simulink model "MICRORRED"  (R2018a)
settings: Solver=FixedStepDiscrete  StartTime=0.0  StopTime=0.7  FixedStep=1/(60*32)  RelTol=1e-3  EnableMultiTasking=on
InitFcn:
  | close
  | clear
  | clc
  | Ts=1/(60*32);
  | run script_client_3_inicio_ti.m
  | set_param('MICRORRED/EMISOR-RECEPTOR/TCP_IP_RX3/ESCRITURA', 'Value','0');
  | set_param('MICRORRED/EMISOR-RECEPTOR/TCP_IP_RX3/RETARDO', 'Value','0');
StopFcn:
  | %run script_graficas.m
undefined symbols (not defined in the file or in its folder): DiscIntNeverNeededParam, Int, Ip1, man, Vuc
libraries: powerlib x15, simulink x6, libreria_medidores3 x2, libreria_comunicaciones_red3 x1
(part 1 of 2)
settings Model: SnapshotInterval=1  Creator=Juan Antonio Ocampo  LastModifiedBy=ana-n
settings DataIOCC: LimitDataPoints=on
settings OptimizationCC: LifeSpan=inf
settings DebuggingCC: AllowSymbolicDim=off  SFUnexpectedBacktrackingDiag=warning  SFNoUnconditionalDefaultTransitionDiag=warning  SFExecutionAtInitializationDiag=none
settings ModelReferenceCC: PropagateSignalLabelsOutOfModel=off
settings CodeAppCC: StateflowObjectComments=on
settings GRTTargetCC: TargetLangStandard=C89/C90 (ANSI)
settings ConfigComp: CovMetricSettings=dw  CovHtmlReporting=on  CovSaveCumulativeToWorkspaceVar=on  CovSaveSingleToWorkspaceVar=on  CovExternalEMLEnable=off
settings SimscapeCC: SimscapeNormalizeSystem=off

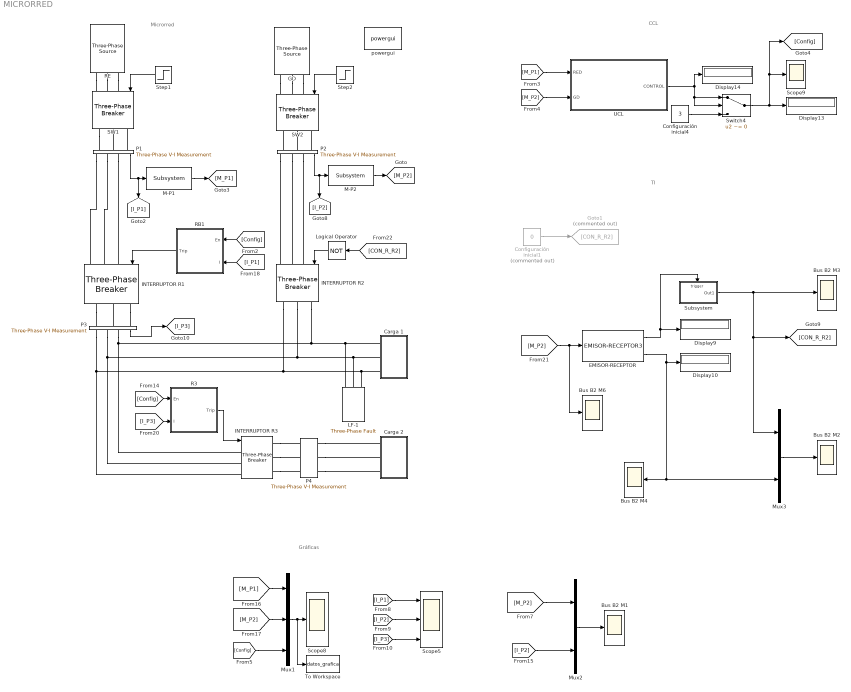
== system MICRORRED ==
  note: Microrred
  note: Gráficas
  note: TI
  note: CCL
  "               LF-1" : powerlib/Elements/Three-Phase Fault  InitialStates=0  FaultA=on  FaultB=on  FaultC=on  GroundFault=on  SwitchTimes=0.4  External=off  SwitchStatus=NaN  FaultResistance=50  GroundResistance=400  SnubberResistance=1e6  SnubberCapacitance=inf  Measurements=Fault currents
  Bus B2 M{1..4,6} (5 alike) : Scope
  Carga 1 : Subsystem
  Carga 2 : Subsystem
  Configuración inicial1 : Constant  Commented=on  Value=0
  Configuración inicial4 : Constant  Value=3
  Display{9..10,13..14} (4 alike) : Display
  EMISOR-RECEPTOR : libreria_comunicaciones_red3/EMISOR-RECEPTOR3  SystemSampleTime=-1
      link override TCP_IP_RX3/ESCRITURA: Value=client_1.dato_lectura
      link override TCP_IP_RX3/RETARDO: Value=e
  GD : powerlib/Electrical Sources/Three-Phase Source  InternalConnection=Yg  VoltagePhases=off  Voltage=13200  PhaseAngle=0  Voltage_phases=[25e3 25e3 25e3]/sqrt(3)  PhaseAngles_phases=[0 -120 +120]  Frequency=60  NonIdealSource=on  SpecifyImpedance=on  Resistance=25^2/1000/10  Inductance=25^2/1000/377  ShortCircuitLevel=100e6  BaseVoltage=13200  XRratio=10  BusType=swing  Pref=1000  Qref=0  Prefabc=[10e3, 10e3, 10e3]  Qrefabc=[0, 0, 0]  Qmin=-inf  Qmax=inf
  Goto1 : Goto  Commented=on  GotoTag=CON_R_R2
  INTERRUPTOR R1 : powerlib/Elements/Three-Phase Breaker  InitialState=closed  SwitchA=on  SwitchB=on  SwitchC=on  SwitchTimes=[20]  External=on  BreakerResistance=0.0000001  SnubberResistance=1e6  SnubberCapacitance=inf  Measurements=None
      link override Breaker A: Measurements=None
      link override Breaker B: Measurements=None
      link override Breaker C: Measurements=None
  INTERRUPTOR R2 : powerlib/Elements/Three-Phase Breaker  InitialState=closed  SwitchA=on  SwitchB=on  SwitchC=on  SwitchTimes=[20]  External=on  BreakerResistance=0.0000001  SnubberResistance=1e6  SnubberCapacitance=inf  Measurements=None
      link override Breaker A: Measurements=None
      link override Breaker B: Measurements=None
      link override Breaker C: Measurements=None
  INTERRUPTOR R3 : powerlib/Elements/Three-Phase Breaker  InitialState=closed  SwitchA=on  SwitchB=on  SwitchC=on  SwitchTimes=[20]  External=on  BreakerResistance=0.0000001  SnubberResistance=1e6  SnubberCapacitance=inf  Measurements=None
      link override Breaker A: Measurements=None
      link override Breaker B: Measurements=None
      link override Breaker C: Measurements=None
  Logical Operator : Logic  Operator=NOT  AllPortsSameDT=off  OutDataTypeStr=fixdt(1,16)
  M-P1 : libreria_medidores3/Subsystem  SystemSampleTime=-1
  M-P2 : libreria_medidores3/Subsystem  SystemSampleTime=-1
  Mux1 : Mux  Inputs=3
  Mux2 : Mux  Inputs=2
  Mux3 : Mux  Inputs=2
  P1 : powerlib/Measurements/Three-Phase V-I Measurement  VoltageMeasurement=no  SetLabelV=off  LabelV=V_P1  Vpu=off  VpuLL=off  CurrentMeasurement=yes  SetLabelI=off  LabelI=I_P1  Ipu=off  Pbase=100e6  Vbase=500e3  OutputType=Complex  PhasorSimulation=off  PSBequivalent=0
  P2 : powerlib/Measurements/Three-Phase V-I Measurement  VoltageMeasurement=no  SetLabelV=on  LabelV=V_P2  Vpu=off  VpuLL=off  CurrentMeasurement=yes  SetLabelI=off  LabelI=I_P2  Ipu=off  Pbase=100e6  Vbase=500e3  OutputType=Complex  PhasorSimulation=off  PSBequivalent=0
  P3 : powerlib/Measurements/Three-Phase V-I Measurement  VoltageMeasurement=no  SetLabelV=off  LabelV=V_P1  Vpu=off  VpuLL=off  CurrentMeasurement=yes  SetLabelI=off  LabelI=I_P1  Ipu=off  Pbase=100e6  Vbase=500e3  OutputType=Complex  PhasorSimulation=off  PSBequivalent=0
  P4 : powerlib/Measurements/Three-Phase V-I Measurement  VoltageMeasurement=phase-to-ground  SetLabelV=on  LabelV=V_P4  Vpu=off  VpuLL=off  CurrentMeasurement=yes  SetLabelI=on  LabelI=I_P4  Ipu=off  Pbase=100e6  Vbase=500e3  OutputType=Complex  PhasorSimulation=off  PSBequivalent=0
  R3 : Subsystem  mask(Proteccion de Sobrecorriente multitopologia){menu=3, TCpopup1=IEC Standard Inverse, k1=0.14, alpha1=0.02, B1=0, PS1=1.15, TMS1=0.04, Tins1=0.05, Esc1=3, TCpopup2=IEC Standard Inverse, k2=0.14, alpha2=0.02, B2=0, PS2=1.15, TMS2=0.03, Tins2=0.05, Esc2=3, TCpopup3=IEC Standard Inverse, k3=0.14, alpha3=0.02, B3=0, PS3=1.15, TMS3=0.01, Tins3=0.03, Esc3=3, Vp=25, Vs=25, F=60}
      mask prompts: menu "Numero de Topologias"; TCpopup1 "Caracteristica de Disparo"; k1 "k"; alpha1 "alpha"; B1 "B"; PS1 "Seteo disparo(PS)/Seteo inferior(I>)"; TMS1 "Multiplicador de Tiempo"; Tins1 "Tins"; Esc1 "Escala"; TCpopup2 "Caracteristica de Disparo"; k2 "k"; alpha2 "alpha"; B2 "B"; PS2 "Seteo disparo(PS)/Seteo inferior(I>)"; TMS2 "Multiplicador de tiempo"; Tins2 "Tins"; Esc2 "Escala"; TCpopup3 "Caracteristica de Disparo"; k3 "k"; alpha3 "alpha"; B3 "B"; PS3 "Seteo disparo(PS)/Seteo inferior(I>)"; TMS3 "Multiplicador de Tiempo"; Tins3 "Tins"; Esc3 "Escala"; Vp "Primario CT"; Vs "Secundario CT"; F "Frecuencia"
      mask help: Proteccion de Sobrecorriente con tres topologias internas controladas por una señal de control externa.
      mask init:
      | warning('off','Simulink:Masking:Invalid_Visible_Flag')
      mask TypeOptions menu: 1 | 2 | 3
      mask Callback menu:
      | h = getSimulinkBlockHandle(gcb);
      | menu1 = get_param(h,'menu');
      | if strcmp(menu1,num2str(1))
      |     set_param(h,'MaskVisibilities',{'on',...
      |         'on','on','on','on','on','on','on','on',...%proteccion 1 activa
      |         'off','off','off','off','off','off','off','off',...%proteccion 2 desactivada
      |         'off','off','off','off','off','off','off','off',...%proteccion 3 desactivada
      |         'on','on','on'});%Otros parametros activados
      |     Int=1;
      | elseif strcmp(menu1,num2str(2))
      |  set_param(h,'MaskVisibilities',{'on',...
      |         'on','on','on','on','on','on','on','on',...%proteccion 1 activa
      |         'on','on','on','on','on','on','on','on',...%proteccion 2 activa
      |         'off','off','off','off','off','off','off','off',...%proteccion 3 desactivada
      |         'on','on','on'});%Otros parametros activados
      |     Int=2;
      | else
      | set_param(h,'MaskVisibilities',{'on',...
      |         'on','on','on','on','on','on','on','on',...%proteccion 1 activa
      |         'on','on','on','on','on','on','on','on',...%proteccion 2 activa
      |         'on','on','on','on','on','on','on','on',...%proteccion 3 desactivada
      |         'on','on','on'});%Otros parametros activados
      |     Int=3;
      | end
      mask TypeOptions TCpopup1: IEC Standard Inverse | IEC Very Inverse | IEC Long Time Inverse | IEC Extremely Inverse | IEC Ultra Inverse | IEEE Moderately Inverse | IEEE Very Inverse | IEEE Extremely Inverse
      mask Callback TCpopup1:
      | switch(get_param(gcb,'TCpopup1'))
      |     case 'IEC Standard Inverse'
      |         set_param(gcb,'k1','0.14');
      |         set_param(gcb,'alpha1','0.02');
      |         set_param(gcb,'B1','0');
      |     case 'IEC Very Inverse'
      |         set_param(gcb,'k1','13.5');
      |         set_param(gcb,'alpha1','1');
      |         set_param(gcb,'B1','0');
      |     case 'IEC Long Time Inverse'
      |         set_param(gcb,'k1','120');
      |         set_param(gcb,'alpha1','1');
      |         set_param(gcb,'B1','0');
      |     case 'IEC Extremely Inverse'
      |         set_param(gcb,'k1','80');
      |         set_param(gcb,'alpha1','2');
      |         set_param(gcb,'B1','0');
      |     case 'IEC Ultra Inverse'
      |         set_param(gcb,'k1','315.2');
      |         set_param(gcb,'alpha1','2.5');
      |         set_param(gcb,'B1','0');
      |     case 'IEEE Moderately Inverse'
      |         set_param(gcb,'k1','0.0515');
      |         set_param(gcb,'alpha1','0.02');
      |         set_param(gcb,'B1','0.114');
      |     case 'IEEE Very Inverse'
      |         set_param(gcb,'k1','19.61');
      |         set_param(gcb,'alpha1','2');
      |         set_param(gcb,'B1','0.491');
      |     case 'IEEE Extremely Inverse'
      |         set_param(gcb,'k1','28.2');
      |         set_param(gcb,'alpha1','2');
      |         set_param(gcb,'B1','0.1217');
      | end
      | % Plotting IDMT Curve
      | clf('reset')
      | TMS = str2num(get_param(gcb,'TMS1'));
      | Vp = str2num(get_param(gcb,'Vp'));
      | PS=str2num(get_param(gcb,'PS1'));
      | k = str2num(get_param(gcb,'k1'));
      | alpha = str2num(get_param(gcb,'alpha1'));
      | B = str2num(get_param(gcb,'B1'));
      | Esc = str2num(get_param(gcb,'Esc1'));
      | Tins = str2num(get_param(gcb,'Tins1'));
      | I = [1.1:0.1:Esc];
      | I1=[Esc,Esc:0.1:30];
      | y=((k./((I.^alpha)-1))+B)*TMS;
      | Tin=[((k./((Esc.^alpha)-1))+B)*TMS,ones(1,length(I1)-1)*Tins];
      | loglog(I,y,'b');
      | hold on
      | loglog(I1,Tin,'b');
      | set(gcf, 'Position', [200 150 300 500]);
      | switch(get_param(gcb,'TCpopup1'))
      |     case 'IEC Standard Inverse'
      |         title('IEC Standard Inverse');
      |     case 'IEC Very Inverse'
      |         title('IEC Very Inverse');
      |     case 'IEC Long Time Inverse'
      |         title('IEC Long Time Inverse');
      |     case 'IEC Extremely Inverse'
      |         title('IEC Extremely Inverse');
      |      case 'IEC Ultra Inverse'
      |         title('IEC Ultra Inverse');
      |     case 'IEEE Moderately Inverse'
      |         title('IEEE Moderately Inverse');
      |     case 'IEEE Very Inverse'
      |         title('IEEE Very Inverse');
      |     case 'IEEE Extremely Inverse'
      |         title('IEEE Extremely Inverse');
      | end
      | ymax=10^ceil(log10(max(y)));
      | set(gca, 'XTick',[1:10 20]);
      | set(gca, 'YTick',[0 ymax/1000 ymax/500 ymax/200 ymax/100 ymax/50 ymax/20 ymax/10 ymax/5 ymax/2 ymax]);
      | xlim([0.9 30]);
      | ylim([0.01 ymax]);
      | xlabel(['Corriente multiplicada por Ipick-up(' num2str(PS*Vp) 'A)']);
      | ylabel('Tiempo de Operacion (Seg)');
      | grid on;
      | set(gca, 'color',[0.9608 0.9608 0.937]);
      | set(gca, 'gridcolor',[0 0.6902 0.3137]);
      mask Callback PS1:
      | % Plotting IDMT Curve
      | clf('reset')
      | TMS = str2num(get_param(gcb,'TMS1'));
      | Vp = str2num(get_param(gcb,'Vp'));
      | PS=str2num(get_param(gcb,'PS1'));
      | k = str2num(get_param(gcb,'k1'));
      | alpha = str2num(get_param(gcb,'alpha1'));
      | B = str2num(get_param(gcb,'B1'));
      | Esc = str2num(get_param(gcb,'Esc1'));
      | Tins = str2num(get_param(gcb,'Tins1'));
      | I = [1.1:0.1:Esc];
      | I1=[Esc,Esc:0.1:30];
      | y=((k./((I.^alpha)-1))+B)*TMS;
      | Tin=[((k./((Esc.^alpha)-1))+B)*TMS,ones(1,length(I1)-1)*Tins];
      | loglog(I,y,'b');
      | hold on
      | loglog(I1,Tin,'b');
      | set(gcf, 'Position', [200 150 300 500]);
      | switch(get_param(gcb,'TCpopup1'))
      |     case 'IEC Standard Inverse'
      |         title('IEC Standard Inverse');
      |     case 'IEC Very Inverse'
      |         title('IEC Very Inverse');
      |     case 'IEC Long Time Inverse'
      |         title('IEC Long Time Inverse');
      |     case 'IEC Extremely Inverse'
      |         title('IEC Extremely Inverse');
      |      case 'IEC Ultra Inverse'
      |         title('IEC Ultra Inverse');
      |     case 'IEEE Moderately Inverse'
      |         title('IEEE Moderately Inverse');
      |     case 'IEEE Very Inverse'
      |         title('IEEE Very Inverse');
      |     case 'IEEE Extremely Inverse'
      |         title('IEEE Extremely Inverse');
      | end
      | ymax=10^ceil(log10(max(y)));
      | set(gca, 'XTick',[1:10 20]);
      | set(gca, 'YTick',[0 ymax/1000 ymax/500 ymax/200 ymax/100 ymax/50 ymax/20 ymax/10 ymax/5 ymax/2 ymax]);
      | xlim([0.9 30]);
      | ylim([0.01 ymax]);
      | xlabel(['Corriente multiplicada por Ipick-up(' num2str(PS*Vp) 'A)']);
      | ylabel('Tiempo de Operacion (Seg)');
      | grid on;
      | set(gca, 'color',[0.9608 0.9608 0.937]);
      | set(gca, 'gridcolor',[0 0.6902 0.3137]);
      mask Callback TMS1:
      | % Plotting IDMT Curve
      | clf('reset')
      | TMS = str2num(get_param(gcb,'TMS1'));
      | Vp = str2num(get_param(gcb,'Vp'));
      | PS=str2num(get_param(gcb,'PS1'));
      | k = str2num(get_param(gcb,'k1'));
      | alpha = str2num(get_param(gcb,'alpha1'));
      | B = str2num(get_param(gcb,'B1'));
      | Esc = str2num(get_param(gcb,'Esc1'));
      | Tins = str2num(get_param(gcb,'Tins1'));
      | I = [1.1:0.1:Esc];
      | I1=[Esc,Esc:0.1:30];
      | y=((k./((I.^alpha)-1))+B)*TMS;
      | Tin=[((k./((Esc.^alpha)-1))+B)*TMS,ones(1,length(I1)-1)*Tins];
      | loglog(I,y,'b');
      | hold on
      | loglog(I1,Tin,'b');
      | set(gcf, 'Position', [200 150 300 500]);
      | switch(get_param(gcb,'TCpopup1'))
      |     case 'IEC Standard Inverse'
      |         title('IEC Standard Inverse');
      |     case 'IEC Very Inverse'
      |         title('IEC Very Inverse');
      |     case 'IEC Long Time Inverse'
      |         title('IEC Long Time Inverse');
      |     case 'IEC Extremely Inverse'
      |         title('IEC Extremely Inverse');
      |      case 'IEC Ultra Inverse'
      |         title('IEC Ultra Inverse');
      |     case 'IEEE Moderately Inverse'
      |         title('IEEE Moderately Inverse');
      |     case 'IEEE Very Inverse'
      |         title('IEEE Very Inverse');
      |     case 'IEEE Extremely Inverse'
      |         title('IEEE Extremely Inverse');
      | end
      | ymax=10^ceil(log10(max(y)));
      | set(gca, 'XTick',[1:10 20]);
      | set(gca, 'YTick',[0 ymax/1000 ymax/500 ymax/200 ymax/100 ymax/50 ymax/20 ymax/10 ymax/5 ymax/2 ymax]);
      | xlim([0.9 30]);
      | ylim([0.01 ymax]);
      | xlabel(['Corriente multiplicada por Ipick-up(' num2str(PS*Vp) 'A)']);
      | ylabel('Tiempo de Operacion (Seg)');
      | grid on;
      | set(gca, 'color',[0.9608 0.9608 0.937]);
      | set(gca, 'gridcolor',[0 0.6902 0.3137]);
      mask Callback Tins1:
      | % Plotting IDMT Curve
      | clf('reset')
      | TMS = str2num(get_param(gcb,'TMS1'));
      | Vp = str2num(get_param(gcb,'Vp'));
      | PS=str2num(get_param(gcb,'PS1'));
      | k = str2num(get_param(gcb,'k1'));
      | alpha = str2num(get_param(gcb,'alpha1'));
      | B = str2num(get_param(gcb,'B1'));
      | Esc = str2num(get_param(gcb,'Esc1'));
      | Tins = str2num(get_param(gcb,'Tins1'));
      | I = [1.1:0.1:Esc];
      | I1=[Esc,Esc:0.1:30];
      | y=((k./((I.^alpha)-1))+B)*TMS;
      | Tin=[((k./((Esc.^alpha)-1))+B)*TMS,ones(1,length(I1)-1)*Tins];
      | loglog(I,y,'b');
      | hold on
      | loglog(I1,Tin,'b');
      | set(gcf, 'Position', [200 150 300 500]);
      | switch(get_param(gcb,'TCpopup1'))
      |     case 'IEC Standard Inverse'
      |         title('IEC Standard Inverse');
      |     case 'IEC Very Inverse'
      |         title('IEC Very Inverse');
      |     case 'IEC Long Time Inverse'
      |         title('IEC Long Time Inverse');
      |     case 'IEC Extremely Inverse'
      |         title('IEC Extremely Inverse');
      |      case 'IEC Ultra Inverse'
      |         title('IEC Ultra Inverse');
      |     case 'IEEE Moderately Inverse'
      |         title('IEEE Moderately Inverse');
      |     case 'IEEE Very Inverse'
      |         title('IEEE Very Inverse');
      |     case 'IEEE Extremely Inverse'
      |         title('IEEE Extremely Inverse');
      | end
      | ymax=10^ceil(log10(max(y)));
      | set(gca, 'XTick',[1:10 20]);
      | set(gca, 'YTick',[0 ymax/1000 ymax/500 ymax/200 ymax/100 ymax/50 ymax/20 ymax/10 ymax/5 ymax/2 ymax]);
      | xlim([0.9 30]);
      | ylim([0.01 ymax]);
      | xlabel(['Corriente multiplicada por Ipick-up(' num2str(PS*Vp) 'A)']);
      | ylabel('Tiempo de Operacion (Seg)');
      | grid on;
      | set(gca, 'color',[0.9608 0.9608 0.937]);
      | set(gca, 'gridcolor',[0 0.6902 0.3137]);
      mask Callback Esc1:
      | % Plotting IDMT Curve
      | clf('reset')
      | TMS = str2num(get_param(gcb,'TMS1'));
      | Vp = str2num(get_param(gcb,'Vp'));
      | PS=str2num(get_param(gcb,'PS1'));
      | k = str2num(get_param(gcb,'k1'));
      | alpha = str2num(get_param(gcb,'alpha1'));
      | B = str2num(get_param(gcb,'B1'));
      | Esc = str2num(get_param(gcb,'Esc1'));
      | Tins = str2num(get_param(gcb,'Tins1'));
      | I = [1.1:0.1:Esc];
      | I1=[Esc,Esc:0.1:30];
      | y=((k./((I.^alpha)-1))+B)*TMS;
      | Tin=[((k./((Esc.^alpha)-1))+B)*TMS,ones(1,length(I1)-1)*Tins];
      | loglog(I,y,'b');
      | hold on
      | loglog(I1,Tin,'b');
      | set(gcf, 'Position', [200 150 300 500]);
      | switch(get_param(gcb,'TCpopup1'))
      |     case 'IEC Standard Inverse'
      |         title('IEC Standard Inverse');
      |     case 'IEC Very Inverse'
      |         title('IEC Very Inverse');
      |     case 'IEC Long Time Inverse'
      |         title('IEC Long Time Inverse');
      |     case 'IEC Extremely Inverse'
      |         title('IEC Extremely Inverse');
      |      case 'IEC Ultra Inverse'
      |         title('IEC Ultra Inverse');
      |     case 'IEEE Moderately Inverse'
      |         title('IEEE Moderately Inverse');
      |     case 'IEEE Very Inverse'
      |         title('IEEE Very Inverse');
      |     case 'IEEE Extremely Inverse'
      |         title('IEEE Extremely Inverse');
      | end
      | ymax=10^ceil(log10(max(y)));
      | set(gca, 'XTick',[1:10 20]);
      | set(gca, 'YTick',[0 ymax/1000 ymax/500 ymax/200 ymax/100 ymax/50 ymax/20 ymax/10 ymax/5 ymax/2 ymax]);
      | xlim([0.9 30]);
      | ylim([0.01 ymax]);
      | xlabel(['Corriente multiplicada por Ipick-up(' num2str(PS*Vp) 'A)']);
      | ylabel('Tiempo de Operacion (Seg)');
      | grid on;
      | set(gca, 'color',[0.9608 0.9608 0.937]);
      | set(gca, 'gridcolor',[0 0.6902 0.3137]);
      mask TypeOptions TCpopup2: IEC Standard Inverse | IEC Very Inverse | IEC Long Time Inverse | IEC Extremely Inverse | IEC Ultra Inverse | IEEE Moderately Inverse | IEEE Very Inverse | IEEE Extremely Inverse
      mask Callback TCpopup2:
      | switch(get_param(gcb,'TCpopup2'))
      |     case 'IEC Standard Inverse'
      |         set_param(gcb,'k2','0.14');
      |         set_param(gcb,'alpha2','0.02');
      |         set_param(gcb,'B2','0');
      |     case 'IEC Very Inverse'
      |         set_param(gcb,'k2','13.5');
      |         set_param(gcb,'alpha2','1');
      |         set_param(gcb,'B2','0');
      |     case 'IEC Long Time Inverse'
      |         set_param(gcb,'k2','120');
      |         set_param(gcb,'alpha2','1');
      |         set_param(gcb,'B2','0');
      |     case 'IEC Extremely Inverse'
      |         set_param(gcb,'k2','80');
      |         set_param(gcb,'alpha2','2');
      |         set_param(gcb,'B2','0');
      |     case 'IEC Ultra Inverse'
      |         set_param(gcb,'k2','315.2');
      |         set_param(gcb,'alpha2','2.5');
      |         set_param(gcb,'B2','0');
      |     case 'IEEE Moderately Inverse'
      |         set_param(gcb,'k2','0.0515');
      |         set_param(gcb,'alpha2','0.02');
      |         set_param(gcb,'B2','0.114');
      |     case 'IEEE Very Inverse'
      |         set_param(gcb,'k2','19.61');
      |         set_param(gcb,'alpha2','2');
      |         set_param(gcb,'B2','0.491');
      |     case 'IEEE Extremely Inverse'
      |         set_param(gcb,'k2','28.2');
      |         set_param(gcb,'alpha2','2');
      |         set_param(gcb,'B2','0.1217');
      | end
      | % Plotting IDMT Curve
      | clf('reset')
      | TMS = str2num(get_param(gcb,'TMS2'));
      | Vp = str2num(get_param(gcb,'Vp'));
      | PS=str2num(get_param(gcb,'PS2'));
      | k = str2num(get_param(gcb,'k2'));
      | alpha = str2num(get_param(gcb,'alpha2'));
      | B = str2num(get_param(gcb,'B2'));
      | Esc = str2num(get_param(gcb,'Esc2'));
      | Tins = str2num(get_param(gcb,'Tins2'));
      | I = [1.1:0.1:Esc];
      | I1=[Esc,Esc:0.1:30];
      | y=((k./((I.^alpha)-1))+B)*TMS;
      | Tin=[((k./((Esc.^alpha)-1))+B)*TMS,ones(1,length(I1)-1)*Tins];
      | loglog(I,y,'r');
      | hold on
      | loglog(I1,Tin,'r');
      | set(gcf, 'Position', [200 150 300 500]);
      | switch(get_param(gcb,'TCpopup2'))
      |     case 'IEC Standard Inverse'
      |         title('IEC Standard Inverse');
      |     case 'IEC Very Inverse'
      |         title('IEC Very Inverse');
      |     case 'IEC Long Time Inverse'
      |         title('IEC Long Time Inverse');
      |     case 'IEC Extremely Inverse'
      |         title('IEC Extremely Inverse');
      |      case 'IEC Ultra Inverse'
      |         title('IEC Ultra Inverse');
      |     case 'IEEE Moderately Inverse'
      |         title('IEEE Moderately Inverse');
      |     case 'IEEE Very Inverse'
      |         title('IEEE Very Inverse');
      |     case 'IEEE Extremely Inverse'
      |         title('IEEE Extremely Inverse');
      | end
      | ymax=10^ceil(log10(max(y)));
      | set(gca, 'XTick',[1:10 20]);
      | set(gca, 'YTick',[0 ymax/1000 ymax/500 ymax/200 ymax/100 ymax/50 ymax/20 ymax/10 ymax/5 ymax/2 ymax]);
      | xlim([0.9 30]);
      | ylim([0.01 ymax]);
      | xlabel(['Corriente multiplicada por Ipick-up(' num2str(PS*Vp) 'A)']);
      | ylabel('Tiempo de Operacion (Seg)');
      | grid on;
      | set(gca, 'color',[0.9608 0.9608 0.937]);
      | set(gca, 'gridcolor',[0 0.6902 0.3137]);
      mask Callback PS2:
      | % Plotting IDMT Curve
      | clf('reset')
      | TMS = str2num(get_param(gcb,'TMS2'));
      | Vp = str2num(get_param(gcb,'Vp'));
      | PS=str2num(get_param(gcb,'PS2'));
      | k = str2num(get_param(gcb,'k2'));
      | alpha = str2num(get_param(gcb,'alpha2'));
      | B = str2num(get_param(gcb,'B2'));
      | Esc = str2num(get_param(gcb,'Esc2'));
      | Tins = str2num(get_param(gcb,'Tins2'));
      | I = [1.1:0.1:Esc];
      | I1=[Esc,Esc:0.1:30];
      | y=((k./((I.^alpha)-1))+B)*TMS;
      | Tin=[((k./((Esc.^alpha)-1))+B)*TMS,ones(1,length(I1)-1)*Tins];
      | loglog(I,y,'r');
      | hold on
      | loglog(I1,Tin,'r');
      | set(gcf, 'Position', [200 150 300 500]);
      | switch(get_param(gcb,'TCpopup2'))
      |     case 'IEC Standard Inverse'
      |         title('IEC Standard Inverse');
      |     case 'IEC Very Inverse'
      |         title('IEC Very Inverse');
      |     case 'IEC Long Time Inverse'
      |         title('IEC Long Time Inverse');
      |     case 'IEC Extremely Inverse'
      |         title('IEC Extremely Inverse');
      |      case 'IEC Ultra Inverse'
      |         title('IEC Ultra Inverse');
      |     case 'IEEE Moderately Inverse'
      |         title('IEEE Moderately Inverse');
      |     case 'IEEE Very Inverse'
      |         title('IEEE Very Inverse');
      |     case 'IEEE Extremely Inverse'
      |         title('IEEE Extremely Inverse');
      | end
      | ymax=10^ceil(log10(max(y)));
      | set(gca, 'XTick',[1:10 20]);
      | set(gca, 'YTick',[0 ymax/1000 ymax/500 ymax/200 ymax/100 ymax/50 ymax/20 ymax/10 ymax/5 ymax/2 ymax]);
      | xlim([0.9 30]);
      | ylim([0.01 ymax]);
      | xlabel(['Corriente multiplicada por Ipick-up(' num2str(PS*Vp) 'A)']);
      | ylabel('Tiempo de Operacion (Seg)');
      | grid on;
      | set(gca, 'color',[0.9608 0.9608 0.937]);
      | set(gca, 'gridcolor',[0 0.6902 0.3137]);
      mask Callback TMS2:
      | % Plotting IDMT Curve
      | clf('reset')
      | TMS = str2num(get_param(gcb,'TMS2'));
      | Vp = str2num(get_param(gcb,'Vp'));
      | PS=str2num(get_param(gcb,'PS2'));
      | k = str2num(get_param(gcb,'k2'));
      | alpha = str2num(get_param(gcb,'alpha2'));
      | B = str2num(get_param(gcb,'B2'));
      | Esc = str2num(get_param(gcb,'Esc2'));
      | Tins = str2num(get_param(gcb,'Tins2'));
      | I = [1.1:0.1:Esc];
      | I1=[Esc,Esc:0.1:30];
      | y=((k./((I.^alpha)-1))+B)*TMS;
      | Tin=[((k./((Esc.^alpha)-1))+B)*TMS,ones(1,length(I1)-1)*Tins];
      | loglog(I,y,'r');
      | hold on
      | loglog(I1,Tin,'r');
      | set(gcf, 'Position', [200 150 300 500]);
      | switch(get_param(gcb,'TCpopup2'))
      |     case 'IEC Standard Inverse'
      |         title('IEC Standard Inverse');
      |     case 'IEC Very Inverse'
      |         title('IEC Very Inverse');
      |     case 'IEC Long Time Inverse'
      |         title('IEC Long Time Inverse');
      |     case 'IEC Extremely Inverse'
      |         title('IEC Extremely Inverse');
      |      case 'IEC Ultra Inverse'
      |         title('IEC Ultra Inverse');
      |     case 'IEEE Moderately Inverse'
      |         title('IEEE Moderately Inverse');
      |     case 'IEEE Very Inverse'
      |         title('IEEE Very Inverse');
      |     case 'IEEE Extremely Inverse'
      |         title('IEEE Extremely Inverse');
      | end
      | ymax=10^ceil(log10(max(y)));
      | set(gca, 'XTick',[1:10 20]);
      | set(gca, 'YTick',[0 ymax/1000 ymax/500 ymax/200 ymax/100 ymax/50 ymax/20 ymax/10 ymax/5 ymax/2 ymax]);
      | xlim([0.9 30]);
      | ylim([0.01 ymax]);
      | xlabel(['Corriente multiplicada por Ipick-up(' num2str(PS*Vp) 'A)']);
      | ylabel('Tiempo de Operacion (Seg)');
      | grid on;
      | set(gca, 'color',[0.9608 0.9608 0.937]);
      | set(gca, 'gridcolor',[0 0.6902 0.3137]);
      mask Callback Tins2:
      | % Plotting IDMT Curve
      | clf('reset')
      | TMS = str2num(get_param(gcb,'TMS2'));
      | Vp = str2num(get_param(gcb,'Vp'));
      | PS=str2num(get_param(gcb,'PS2'));
      | k = str2num(get_param(gcb,'k2'));
      | alpha = str2num(get_param(gcb,'alpha2'));
      | B = str2num(get_param(gcb,'B2'));
      | Esc = str2num(get_param(gcb,'Esc2'));
      | Tins = str2num(get_param(gcb,'Tins2'));
      | I = [1.1:0.1:Esc];
      | I1=[Esc,Esc:0.1:30];
      | y=((k./((I.^alpha)-1))+B)*TMS;
      | Tin=[((k./((Esc.^alpha)-1))+B)*TMS,ones(1,length(I1)-1)*Tins];
      | loglog(I,y,'r');
      | hold on
      | loglog(I1,Tin,'r');
      | set(gcf, 'Position', [200 150 300 500]);
      | switch(get_param(gcb,'TCpopup2'))
      |     case 'IEC Standard Inverse'
      |         title('IEC Standard Inverse');
      |     case 'IEC Very Inverse'
      |         title('IEC Very Inverse');
      |     case 'IEC Long Time Inverse'
      |         title('IEC Long Time Inverse');
      |     case 'IEC Extremely Inverse'
      |         title('IEC Extremely Inverse');
      |      case 'IEC Ultra Inverse'
      |         title('IEC Ultra Inverse');
      |     case 'IEEE Moderately Inverse'
      |         title('IEEE Moderately Inverse');
      |     case 'IEEE Very Inverse'
      |         title('IEEE Very Inverse');
      |     case 'IEEE Extremely Inverse'
      |         title('IEEE Extremely Inverse');
      | end
      | ymax=10^ceil(log10(max(y)));
      | set(gca, 'XTick',[1:10 20]);
      | set(gca, 'YTick',[0 ymax/1000 ymax/500 ymax/200 ymax/100 ymax/50 ymax/20 ymax/10 ymax/5 ymax/2 ymax]);
      | xlim([0.9 30]);
      | ylim([0.01 ymax]);
      | xlabel(['Corriente multiplicada por Ipick-up(' num2str(PS*Vp) 'A)']);
      | ylabel('Tiempo de Operacion (Seg)');
      | grid on;
      | set(gca, 'color',[0.9608 0.9608 0.937]);
      | set(gca, 'gridcolor',[0 0.6902 0.3137]);
      mask Callback Esc2:
      | % Plotting IDMT Curve
      | clf('reset')
      | TMS = str2num(get_param(gcb,'TMS2'));
      | Vp = str2num(get_param(gcb,'Vp'));
      | PS=str2num(get_param(gcb,'PS2'));
      | k = str2num(get_param(gcb,'k2'));
      | alpha = str2num(get_param(gcb,'alpha2'));
      | B = str2num(get_param(gcb,'B2'));
      | Esc = str2num(get_param(gcb,'Esc2'));
      | Tins = str2num(get_param(gcb,'Tins2'));
      | I = [1.1:0.1:Esc];
      | I1=[Esc,Esc:0.1:30];
      | y=((k./((I.^alpha)-1))+B)*TMS;
      | Tin=[((k./((Esc.^alpha)-1))+B)*TMS,ones(1,length(I1)-1)*Tins];
      | loglog(I,y,'r');
      | hold on
      | loglog(I1,Tin,'r');
      | set(gcf, 'Position', [200 150 300 500]);
      | switch(get_param(gcb,'TCpopup2'))
      |     case 'IEC Standard Inverse'
      |         title('IEC Standard Inverse');
      |     case 'IEC Very Inverse'
      |         title('IEC Very Inverse');
      |     case 'IEC Long Time Inverse'
      |         title('IEC Long Time Inverse');
      |     case 'IEC Extremely Inverse'
      |         title('IEC Extremely Inverse');
      |      case 'IEC Ultra Inverse'
      |         title('IEC Ultra Inverse');
      |     case 'IEEE Moderately Inverse'
      |         title('IEEE Moderately Inverse');
      |     case 'IEEE Very Inverse'
      |         title('IEEE Very Inverse');
      |     case 'IEEE Extremely Inverse'
      |         title('IEEE Extremely Inverse');
      | end
      | ymax=10^ceil(log10(max(y)));
      | set(gca, 'XTick',[1:10 20]);
      | set(gca, 'YTick',[0 ymax/1000 ymax/500 ymax/200 ymax/100 ymax/50 ymax/20 ymax/10 ymax/5 ymax/2 ymax]);
      | xlim([0.9 30]);
      | ylim([0.01 ymax]);
      | xlabel(['Corriente multiplicada por Ipick-up(' num2str(PS*Vp) 'A)']);
      | ylabel('Tiempo de Operacion (Seg)');
      | grid on;
      | set(gca, 'color',[0.9608 0.9608 0.937]);
      | set(gca, 'gridcolor',[0 0.6902 0.3137]);
      mask TypeOptions TCpopup3: IEC Standard Inverse | IEC Very Inverse | IEC Long Time Inverse | IEC Extremely Inverse | IEC Ultra Inverse | IEEE Moderately Inverse | IEEE Very Inverse | IEEE Extremely Inverse
      mask Callback TCpopup3:
      | switch(get_param(gcb,'TCpopup3'))
      |     case 'IEC Standard Inverse'
      |         set_param(gcb,'k3','0.14');
      |         set_param(gcb,'alpha3','0.02');
      |         set_param(gcb,'B3','0');
      |     case 'IEC Very Inverse'
      |         set_param(gcb,'k3','13.5');
      |         set_param(gcb,'alpha3','1');
      |         set_param(gcb,'B3','0');
      |     case 'IEC Long Time Inverse'
      |         set_param(gcb,'k3','120');
      |         set_param(gcb,'alpha3','1');
      |         set_param(gcb,'B3','0');
      |     case 'IEC Extremely Inverse'
      |         set_param(gcb,'k3','80');
      |         set_param(gcb,'alpha3','2');
      |         set_param(gcb,'B3','0');
      |     case 'IEC Ultra Inverse'
      |         set_param(gcb,'k3','315.2');
      |         set_param(gcb,'alpha3','2.5');
      |         set_param(gcb,'B3','0');
      |     case 'IEEE Moderately Inverse'
      |         set_param(gcb,'k3','0.0515');
      |         set_param(gcb,'alpha3','0.02');
      |         set_param(gcb,'B3','0.114');
      |     case 'IEEE Very Inverse'
      |         set_param(gcb,'k3','19.61');
      |         set_param(gcb,'alpha3','2');
      |         set_param(gcb,'B3','0.491');
      |     case 'IEEE Extremely Inverse'
      |         set_param(gcb,'k3','28.2');
      |         set_param(gcb,'alpha3','2');
      |         set_param(gcb,'B3','0.1217');
      | end
      | % Plotting IDMT Curve
      | clf('reset')
      | TMS = str2num(get_param(gcb,'TMS3'));
      | Vp = str2num(get_param(gcb,'Vp'));
      | PS=str2num(get_param(gcb,'PS3'));
      | k = str2num(get_param(gcb,'k3'));
      | alpha = str2num(get_param(gcb,'alpha3'));
      | B = str2num(get_param(gcb,'B3'));
      | Esc = str2num(get_param(gcb,'Esc3'));
      | Tins = str2num(get_param(gcb,'Tins3'));
      | I = [1.1:0.1:Esc];
      | I1=[Esc,Esc:0.1:30];
      | y=((k./((I.^alpha)-1))+B)*TMS;
      | Tin=[((k./((Esc.^alpha)-1))+B)*TMS,ones(1,length(I1)-1)*Tins];
      | loglog(I,y,'m');
      | hold on
      | loglog(I1,Tin,'m');
      | set(gcf, 'Position', [200 150 300 500]);
      | switch(get_param(gcb,'TCpopup3'))
      |     case 'IEC Standard Inverse'
      |         title('IEC Standard Inverse');
      |     case 'IEC Very Inverse'
      |         title('IEC Very Inverse');
      |     case 'IEC Long Time Inverse'
      |         title('IEC Long Time Inverse');
      |     case 'IEC Extremely Inverse'
      |         title('IEC Extremely Inverse');
      |      case 'IEC Ultra Inverse'
      |         title('IEC Ultra Inverse');
      |     case 'IEEE Moderately Inverse'
      |         title('IEEE Moderately Inverse');
      |     case 'IEEE Very Inverse'
      |         title('IEEE Very Inverse');
      |     case 'IEEE Extremely Inverse'
      |         title('IEEE Extremely Inverse');
      | end
      | ymax=10^ceil(log10(max(y)));
      | set(gca, 'XTick',[1:10 20]);
      | set(gca, 'YTick',[0 ymax/1000 ymax/500 ymax/200 ymax/100 ymax/50 ymax/20 ymax/10 ymax/5 ymax/2 ymax]);
      | xlim([0.9 30]);
      | ylim([0.01 ymax]);
      | xlabel(['Corriente multiplicada por Ipick-up(' num2str(PS*Vp) 'A)']);
      | ylabel('Tiempo de Operacion (Seg)');
      | grid on;
      | set(gca, 'color',[0.9608 0.9608 0.937]);
      | set(gca, 'gridcolor',[0 0.6902 0.3137]);
      mask Callback PS3:
      | % Plotting IDMT Curve
      | clf('reset')
      | TMS = str2num(get_param(gcb,'TMS3'));
      | Vp = str2num(get_param(gcb,'Vp'));
      | PS=str2num(get_param(gcb,'PS3'));
      | k = str2num(get_param(gcb,'k3'));
      | alpha = str2num(get_param(gcb,'alpha3'));
      | B = str2num(get_param(gcb,'B3'));
      | Esc = str2num(get_param(gcb,'Esc3'));
      | Tins = str2num(get_param(gcb,'Tins3'));
      | I = [1.1:0.1:Esc];
      | I1=[Esc,Esc:0.1:30];
      | y=((k./((I.^alpha)-1))+B)*TMS;
      | Tin=[((k./((Esc.^alpha)-1))+B)*TMS,ones(1,length(I1)-1)*Tins];
      | loglog(I,y,'m');
      | hold on
      | loglog(I1,Tin,'m');
      | set(gcf, 'Position', [200 150 300 500]);
      | switch(get_param(gcb,'TCpopup3'))
      |     case 'IEC Standard Inverse'
      |         title('IEC Standard Inverse');
      |     case 'IEC Very Inverse'
      |         title('IEC Very Inverse');
      |     case 'IEC Long Time Inverse'
      |         title('IEC Long Time Inverse');
      |     case 'IEC Extremely Inverse'
      |         title('IEC Extremely Inverse');
      |      case 'IEC Ultra Inverse'
      |         title('IEC Ultra Inverse');
      |     case 'IEEE Moderately Inverse'
      |         title('IEEE Moderately Inverse');
      |     case 'IEEE Very Inverse'
      |         title('IEEE Very Inverse');
      |     case 'IEEE Extremely Inverse'
      |         title('IEEE Extremely Inverse');
      | end
      | ymax=10^ceil(log10(max(y)));
      | set(gca, 'XTick',[1:10 20]);
      | set(gca, 'YTick',[0 ymax/1000 ymax/500 ymax/200 ymax/100 ymax/50 ymax/20 ymax/10 ymax/5 ymax/2 ymax]);
      | xlim([0.9 30]);
      | ylim([0.01 ymax]);
      | xlabel(['Corriente multiplicada por Ipick-up(' num2str(PS*Vp) 'A)']);
      | ylabel('Tiempo de Operacion (Seg)');
      | grid on;
      | set(gca, 'color',[0.9608 0.9608 0.937]);
      | set(gca, 'gridcolor',[0 0.6902 0.3137]);
      mask Callback TMS3:
      | % Plotting IDMT Curve
      | clf('reset')
      | TMS = str2num(get_param(gcb,'TMS3'));
      | Vp = str2num(get_param(gcb,'Vp'));
      | PS=str2num(get_param(gcb,'PS3'));
      | k = str2num(get_param(gcb,'k3'));
      | alpha = str2num(get_param(gcb,'alpha3'));
      | B = str2num(get_param(gcb,'B3'));
      | Esc = str2num(get_param(gcb,'Esc3'));
      | Tins = str2num(get_param(gcb,'Tins3'));
      | I = [1.1:0.1:Esc];
      | I1=[Esc,Esc:0.1:30];
      | y=((k./((I.^alpha)-1))+B)*TMS;
      | Tin=[((k./((Esc.^alpha)-1))+B)*TMS,ones(1,length(I1)-1)*Tins];
      | loglog(I,y,'m');
      | hold on
      | loglog(I1,Tin,'m');
      | set(gcf, 'Position', [200 150 300 500]);
      | switch(get_param(gcb,'TCpopup3'))
      |     case 'IEC Standard Inverse'
      |         title('IEC Standard Inverse');
      |     case 'IEC Very Inverse'
      |         title('IEC Very Inverse');
      |     case 'IEC Long Time Inverse'
      |         title('IEC Long Time Inverse');
      |     case 'IEC Extremely Inverse'
      |         title('IEC Extremely Inverse');
      |      case 'IEC Ultra Inverse'
      |         title('IEC Ultra Inverse');
      |     case 'IEEE Moderately Inverse'
      |         title('IEEE Moderately Inverse');
      |     case 'IEEE Very Inverse'
      |         title('IEEE Very Inverse');
      |     case 'IEEE Extremely Inverse'
      |         title('IEEE Extremely Inverse');
      | end
      | ymax=10^ceil(log10(max(y)));
      | set(gca, 'XTick',[1:10 20]);
      | set(gca, 'YTick',[0 ymax/1000 ymax/500 ymax/200 ymax/100 ymax/50 ymax/20 ymax/10 ymax/5 ymax/2 ymax]);
      | xlim([0.9 30]);
      | ylim([0.01 ymax]);
      | xlabel(['Corriente multiplicada por Ipick-up(' num2str(PS*Vp) 'A)']);
      | ylabel('Tiempo de Operacion (Seg)');
      | grid on;
      | set(gca, 'color',[0.9608 0.9608 0.937]);
      | set(gca, 'gridcolor',[0 0.6902 0.3137]);
      mask Callback Tins3:
      | % Plotting IDMT Curve
      | clf('reset')
      | TMS = str2num(get_param(gcb,'TMS3'));
      | Vp = str2num(get_param(gcb,'Vp'));
      | PS=str2num(get_param(gcb,'PS3'));
      | k = str2num(get_param(gcb,'k3'));
      | alpha = str2num(get_param(gcb,'alpha3'));
      | B = str2num(get_param(gcb,'B3'));
      | Esc = str2num(get_param(gcb,'Esc3'));
      | Tins = str2num(get_param(gcb,'Tins3'));
      | I = [1.1:0.1:Esc];
      | I1=[Esc,Esc:0.1:30];
      | y=((k./((I.^alpha)-1))+B)*TMS;
      | Tin=[((k./((Esc.^alpha)-1))+B)*TMS,ones(1,length(I1)-1)*Tins];
      | loglog(I,y,'m');
      | hold on
      | loglog(I1,Tin,'m');
      | set(gcf, 'Position', [200 150 300 500]);
      | switch(get_param(gcb,'TCpopup3'))
      |     case 'IEC Standard Inverse'
      |         title('IEC Standard Inverse');
      |     case 'IEC Very Inverse'
      |         title('IEC Very Inverse');
      |     case 'IEC Long Time Inverse'
      |         title('IEC Long Time Inverse');
      |     case 'IEC Extremely Inverse'
      |         title('IEC Extremely Inverse');
      |      case 'IEC Ultra Inverse'
      |         title('IEC Ultra Inverse');
      |     case 'IEEE Moderately Inverse'
      |         title('IEEE Moderately Inverse');
      |     case 'IEEE Very Inverse'
      |         title('IEEE Very Inverse');
      |     case 'IEEE Extremely Inverse'
      |         title('IEEE Extremely Inverse');
      | end
      | ymax=10^ceil(log10(max(y)));
      | set(gca, 'XTick',[1:10 20]);
      | set(gca, 'YTick',[0 ymax/1000 ymax/500 ymax/200 ymax/100 ymax/50 ymax/20 ymax/10 ymax/5 ymax/2 ymax]);
      | xlim([0.9 30]);
      | ylim([0.01 ymax]);
      | xlabel(['Corriente multiplicada por Ipick-up(' num2str(PS*Vp) 'A)']);
      | ylabel('Tiempo de Operacion (Seg)');
      | grid on;
      | set(gca, 'color',[0.9608 0.9608 0.937]);
      | set(gca, 'gridcolor',[0 0.6902 0.3137]);
      mask Callback Esc3:
      | % Plotting IDMT Curve
      | clf('reset')
      | TMS = str2num(get_param(gcb,'TMS3'));
      | Vp = str2num(get_param(gcb,'Vp'));
      | PS=str2num(get_param(gcb,'PS3'));
      | k = str2num(get_param(gcb,'k3'));
      | alpha = str2num(get_param(gcb,'alpha3'));
      | B = str2num(get_param(gcb,'B3'));
      | Esc = str2num(get_param(gcb,'Esc3'));
      | Tins = str2num(get_param(gcb,'Tins3'));
      | I = [1.1:0.1:Esc];
      | I1=[Esc,Esc:0.1:30];
      | y=((k./((I.^alpha)-1))+B)*TMS;
      | Tin=[((k./((Esc.^alpha)-1))+B)*TMS,ones(1,length(I1)-1)*Tins];
      | loglog(I,y,'m');
      | hold on
      | loglog(I1,Tin,'m');
      | set(gcf, 'Position', [200 150 300 500]);
      | switch(get_param(gcb,'TCpopup3'))
      |     case 'IEC Standard Inverse'
      |         title('IEC Standard Inverse');
      |     case 'IEC Very Inverse'
      |         title('IEC Very Inverse');
      |     case 'IEC Long Time Inverse'
      |         title('IEC Long Time Inverse');
      |     case 'IEC Extremely Inverse'
      |         title('IEC Extremely Inverse');
      |      case 'IEC Ultra Inverse'
      |         title('IEC Ultra Inverse');
      |     case 'IEEE Moderately Inverse'
      |         title('IEEE Moderately Inverse');
      |     case 'IEEE Very Inverse'
      |         title('IEEE Very Inverse');
      |     case 'IEEE Extremely Inverse'
      |         title('IEEE Extremely Inverse');
      | end
      | ymax=10^ceil(log10(max(y)));
      | set(gca, 'XTick',[1:10 20]);
      | set(gca, 'YTick',[0 ymax/1000 ymax/500 ymax/200 ymax/100 ymax/50 ymax/20 ymax/10 ymax/5 ymax/2 ymax]);
      | xlim([0.9 30]);
      | ylim([0.01 ymax]);
      | xlabel(['Corriente multiplicada por Ipick-up(' num2str(PS*Vp) 'A)']);
      | ylabel('Tiempo de Operacion (Seg)');
      | grid on;
      | set(gca, 'color',[0.9608 0.9608 0.937]);
      | set(gca, 'gridcolor',[0 0.6902 0.3137]);
      mask DialogControl Container6 Prompt: Protecciones
      mask DialogControl Container8 Prompt: Topologia 1
      mask DialogControl Container9 Prompt: Proteccion 51
      mask DialogControl Container10 Prompt: Proteccion 50
      mask DialogControl Container8_copy Prompt: Topologia 2
      mask DialogControl Container9_copy Prompt: Proteccion 51
      mask DialogControl Container10_copy Prompt: Proteccion 50
      mask DialogControl Container8_copy_copy Prompt: Topologia 3
      mask DialogControl Container9_copy_copy Prompt: Proteccion 51
      mask DialogControl Container10_copy_copy Prompt: Proteccion 50
      mask DialogControl Container17 Prompt: Caracteristicas Trafo Corriente
      mask Display:
      | port_label('input',1,'D');
      | port_label('input',2,'I');
      | port_label('output',1,'S');
      | text(0.62, 0.5,'50', 'horizontalAlignment', 'center');
      | text(0.62, 0.3,'51', 'horizontalAlignment', 'center');
      | plot([0.08:0.01:0.32]+0.4,[0:0.01:0.24]*0+0.40);
      | plot(0.25*sin([0:pi/20:2*pi])+0.6,0.25*cos([0:pi/20:2*pi])+0.4);
      | %Linea Salida
      | plot([0.85:0.01:1],[0:0.01:0.15]*0+0.4);
      | %Linea Corriente
      | plot([0.2:0.01:0.35],[0:0.01:0.15]*0+0.4);
      | plot([0.1:0.01:0.2],[0:0.01:0.1]*0+0.15);
      | plot([0.1:0.01:0.35]*0+0.2,[0:0.01:0.25]+0.15);
      | %Linea tension
      | plot([0.15:0.01:0.6],[0:0.01:0.45]*0+0.7);
      | plot([0:0.01:0.05]*0+0.6,[0:0.01:0.05]+0.65);
  RB1 : Subsystem  mask(Proteccion de Sobrecorriente multitopologia){menu=3, TCpopup1=IEC Standard Inverse, k1=0.14, alpha1=0.02, B1=0, PS1=1.15, TMS1=0.045, Tins1=0.25, Esc1=3, TCpopup2=IEC Standard Inverse, k2=0.14, alpha2=0.02, B2=0, PS2=2, TMS2=1, Tins2=10, Esc2=100, TCpopup3=IEC Standard Inverse, k3=0.14, alpha3=0.02, B3=0, PS3=0.9, TMS3=0.02, Tins3=0.09, Esc3=4, Vp=40, Vs=40, F=60}
      mask prompts: menu "Numero de Topologias"; TCpopup1 "Caracteristica de Disparo"; k1 "k"; alpha1 "alpha"; B1 "B"; PS1 "Seteo disparo(PS)/Seteo inferior(I>)"; TMS1 "Multiplicador de Tiempo"; Tins1 "Tins"; Esc1 "Escala"; TCpopup2 "Caracteristica de Disparo"; k2 "k"; alpha2 "alpha"; B2 "B"; PS2 "Seteo disparo(PS)/Seteo inferior(I>)"; TMS2 "Multiplicador de tiempo"; Tins2 "Tins"; Esc2 "Escala"; TCpopup3 "Caracteristica de Disparo"; k3 "k"; alpha3 "alpha"; B3 "B"; PS3 "Seteo disparo(PS)/Seteo inferior(I>)"; TMS3 "Multiplicador de Tiempo"; Tins3 "Tins"; Esc3 "Escala"; Vp "Primario CT"; Vs "Secundario CT"; F "Frecuencia"
      mask help: Proteccion de Sobrecorriente con tres topologias internas controladas por una señal de control externa.
      mask init:
      | warning('off','Simulink:Masking:Invalid_Visible_Flag')
      mask TypeOptions menu: 1 | 2 | 3
      mask Callback menu:
      | h = getSimulinkBlockHandle(gcb);
      | menu1 = get_param(h,'menu');
      | if strcmp(menu1,num2str(1))
      |     set_param(h,'MaskVisibilities',{'on',...
      |         'on','on','on','on','on','on','on','on',...%proteccion 1 activa
      |         'off','off','off','off','off','off','off','off',...%proteccion 2 desactivada
      |         'off','off','off','off','off','off','off','off',...%proteccion 3 desactivada
      |         'on','on','on'});%Otros parametros activados
      |     Int=1;
      | elseif strcmp(menu1,num2str(2))
      |  set_param(h,'MaskVisibilities',{'on',...
      |         'on','on','on','on','on','on','on','on',...%proteccion 1 activa
      |         'on','on','on','on','on','on','on','on',...%proteccion 2 activa
      |         'off','off','off','off','off','off','off','off',...%proteccion 3 desactivada
      |         'on','on','on'});%Otros parametros activados
      |     Int=2;
      | else
      | set_param(h,'MaskVisibilities',{'on',...
      |         'on','on','on','on','on','on','on','on',...%proteccion 1 activa
      |         'on','on','on','on','on','on','on','on',...%proteccion 2 activa
      |         'on','on','on','on','on','on','on','on',...%proteccion 3 desactivada
      |         'on','on','on'});%Otros parametros activados
      |     Int=3;
      | end
      mask TypeOptions TCpopup1: IEC Standard Inverse | IEC Very Inverse | IEC Long Time Inverse | IEC Extremely Inverse | IEC Ultra Inverse | IEEE Moderately Inverse | IEEE Very Inverse | IEEE Extremely Inverse
      mask Callback TCpopup1:
      | switch(get_param(gcb,'TCpopup1'))
      |     case 'IEC Standard Inverse'
      |         set_param(gcb,'k1','0.14');
      |         set_param(gcb,'alpha1','0.02');
      |         set_param(gcb,'B1','0');
      |     case 'IEC Very Inverse'
      |         set_param(gcb,'k1','13.5');
      |         set_param(gcb,'alpha1','1');
      |         set_param(gcb,'B1','0');
      |     case 'IEC Long Time Inverse'
      |         set_param(gcb,'k1','120');
      |         set_param(gcb,'alpha1','1');
      |         set_param(gcb,'B1','0');
      |     case 'IEC Extremely Inverse'
      |         set_param(gcb,'k1','80');
      |         set_param(gcb,'alpha1','2');
      |         set_param(gcb,'B1','0');
      |     case 'IEC Ultra Inverse'
      |         set_param(gcb,'k1','315.2');
      |         set_param(gcb,'alpha1','2.5');
      |         set_param(gcb,'B1','0');
      |     case 'IEEE Moderately Inverse'
      |         set_param(gcb,'k1','0.0515');
      |         set_param(gcb,'alpha1','0.02');
      |         set_param(gcb,'B1','0.114');
      |     case 'IEEE Very Inverse'
      |         set_param(gcb,'k1','19.61');
      |         set_param(gcb,'alpha1','2');
      |         set_param(gcb,'B1','0.491');
      |     case 'IEEE Extremely Inverse'
      |         set_param(gcb,'k1','28.2');
      |         set_param(gcb,'alpha1','2');
      |         set_param(gcb,'B1','0.1217');
      | end
      | % Plotting IDMT Curve
      | clf('reset')
      | TMS = str2num(get_param(gcb,'TMS1'));
      | Vp = str2num(get_param(gcb,'Vp'));
      | PS=str2num(get_param(gcb,'PS1'));
      | k = str2num(get_param(gcb,'k1'));
      | alpha = str2num(get_param(gcb,'alpha1'));
      | B = str2num(get_param(gcb,'B1'));
      | Esc = str2num(get_param(gcb,'Esc1'));
      | Tins = str2num(get_param(gcb,'Tins1'));
      | I = [1.1:0.1:Esc];
      | I1=[Esc,Esc:0.1:30];
      | y=((k./((I.^alpha)-1))+B)*TMS;
      | Tin=[((k./((Esc.^alpha)-1))+B)*TMS,ones(1,length(I1)-1)*Tins];
      | loglog(I,y,'b');
      | hold on
      | loglog(I1,Tin,'b');
      | set(gcf, 'Position', [200 150 300 500]);
      | switch(get_param(gcb,'TCpopup1'))
      |     case 'IEC Standard Inverse'
      |         title('IEC Standard Inverse');
      |     case 'IEC Very Inverse'
      |         title('IEC Very Inverse');
      |     case 'IEC Long Time Inverse'
      |         title('IEC Long Time Inverse');
      |     case 'IEC Extremely Inverse'
      |         title('IEC Extremely Inverse');
      |      case 'IEC Ultra Inverse'
      |         title('IEC Ultra Inverse');
      |     case 'IEEE Moderately Inverse'
      |         title('IEEE Moderately Inverse');
      |     case 'IEEE Very Inverse'
      |         title('IEEE Very Inverse');
      |     case 'IEEE Extremely Inverse'
      |         title('IEEE Extremely Inverse');
      | end
      | ymax=10^ceil(log10(max(y)));
      | set(gca, 'XTick',[1:10 20]);
      | set(gca, 'YTick',[0 ymax/1000 ymax/500 ymax/200 ymax/100 ymax/50 ymax/20 ymax/10 ymax/5 ymax/2 ymax]);
      | xlim([0.9 30]);
      | ylim([0.01 ymax]);
      | xlabel(['Corriente multiplicada por Ipick-up(' num2str(PS*Vp) 'A)']);
      | ylabel('Tiempo de Operacion (Seg)');
      | grid on;
      | set(gca, 'color',[0.9608 0.9608 0.937]);
      | set(gca, 'gridcolor',[0 0.6902 0.3137]);
      mask Callback PS1:
      | % Plotting IDMT Curve
      | clf('reset')
      | TMS = str2num(get_param(gcb,'TMS1'));
      | Vp = str2num(get_param(gcb,'Vp'));
      | PS=str2num(get_param(gcb,'PS1'));
      | k = str2num(get_param(gcb,'k1'));
      | alpha = str2num(get_param(gcb,'alpha1'));
      | B = str2num(get_param(gcb,'B1'));
      | Esc = str2num(get_param(gcb,'Esc1'));
      | Tins = str2num(get_param(gcb,'Tins1'));
      | I = [1.1:0.1:Esc];
      | I1=[Esc,Esc:0.1:30];
      | y=((k./((I.^alpha)-1))+B)*TMS;
      | Tin=[((k./((Esc.^alpha)-1))+B)*TMS,ones(1,length(I1)-1)*Tins];
      | loglog(I,y,'b');
      | hold on
      | loglog(I1,Tin,'b');
      | set(gcf, 'Position', [200 150 300 500]);
      | switch(get_param(gcb,'TCpopup1'))
      |     case 'IEC Standard Inverse'
      |         title('IEC Standard Inverse');
      |     case 'IEC Very Inverse'
      |         title('IEC Very Inverse');
      |     case 'IEC Long Time Inverse'
      |         title('IEC Long Time Inverse');
      |     case 'IEC Extremely Inverse'
      |         title('IEC Extremely Inverse');
      |      case 'IEC Ultra Inverse'
      |         title('IEC Ultra Inverse');
      |     case 'IEEE Moderately Inverse'
      |         title('IEEE Moderately Inverse');
      |     case 'IEEE Very Inverse'
      |         title('IEEE Very Inverse');
      |     case 'IEEE Extremely Inverse'
      |         title('IEEE Extremely Inverse');
      | end
      | ymax=10^ceil(log10(max(y)));
      | set(gca, 'XTick',[1:10 20]);
      | set(gca, 'YTick',[0 ymax/1000 ymax/500 ymax/200 ymax/100 ymax/50 ymax/20 ymax/10 ymax/5 ymax/2 ymax]);
      | xlim([0.9 30]);
      | ylim([0.01 ymax]);
      | xlabel(['Corriente multiplicada por Ipick-up(' num2str(PS*Vp) 'A)']);
      | ylabel('Tiempo de Operacion (Seg)');
      | grid on;
      | set(gca, 'color',[0.9608 0.9608 0.937]);
      | set(gca, 'gridcolor',[0 0.6902 0.3137]);
      mask Callback TMS1:
      | % Plotting IDMT Curve
      | clf('reset')
      | TMS = str2num(get_param(gcb,'TMS1'));
      | Vp = str2num(get_param(gcb,'Vp'));
      | PS=str2num(get_param(gcb,'PS1'));
      | k = str2num(get_param(gcb,'k1'));
      | alpha = str2num(get_param(gcb,'alpha1'));
      | B = str2num(get_param(gcb,'B1'));
      | Esc = str2num(get_param(gcb,'Esc1'));
      | Tins = str2num(get_param(gcb,'Tins1'));
      | I = [1.1:0.1:Esc];
      | I1=[Esc,Esc:0.1:30];
      | y=((k./((I.^alpha)-1))+B)*TMS;
      | Tin=[((k./((Esc.^alpha)-1))+B)*TMS,ones(1,length(I1)-1)*Tins];
      | loglog(I,y,'b');
      | hold on
      | loglog(I1,Tin,'b');
      | set(gcf, 'Position', [200 150 300 500]);
      | switch(get_param(gcb,'TCpopup1'))
      |     case 'IEC Standard Inverse'
      |         title('IEC Standard Inverse');
      |     case 'IEC Very Inverse'
      |         title('IEC Very Inverse');
      |     case 'IEC Long Time Inverse'
      |         title('IEC Long Time Inverse');
      |     case 'IEC Extremely Inverse'
      |         title('IEC Extremely Inverse');
      |      case 'IEC Ultra Inverse'
      |         title('IEC Ultra Inverse');
      |     case 'IEEE Moderately Inverse'
      |         title('IEEE Moderately Inverse');
      |     case 'IEEE Very Inverse'
      |         title('IEEE Very Inverse');
      |     case 'IEEE Extremely Inverse'
      |         title('IEEE Extremely Inverse');
      | end
      | ymax=10^ceil(log10(max(y)));
      | set(gca, 'XTick',[1:10 20]);
      | set(gca, 'YTick',[0 ymax/1000 ymax/500 ymax/200 ymax/100 ymax/50 ymax/20 ymax/10 ymax/5 ymax/2 ymax]);
      | xlim([0.9 30]);
      | ylim([0.01 ymax]);
      | xlabel(['Corriente multiplicada por Ipick-up(' num2str(PS*Vp) 'A)']);
      | ylabel('Tiempo de Operacion (Seg)');
      | grid on;
      | set(gca, 'color',[0.9608 0.9608 0.937]);
      | set(gca, 'gridcolor',[0 0.6902 0.3137]);
      mask Callback Tins1:
      | % Plotting IDMT Curve
      | clf('reset')
      | TMS = str2num(get_param(gcb,'TMS1'));
      | Vp = str2num(get_param(gcb,'Vp'));
      | PS=str2num(get_param(gcb,'PS1'));
      | k = str2num(get_param(gcb,'k1'));
      | alpha = str2num(get_param(gcb,'alpha1'));
      | B = str2num(get_param(gcb,'B1'));
      | Esc = str2num(get_param(gcb,'Esc1'));
      | Tins = str2num(get_param(gcb,'Tins1'));
      | I = [1.1:0.1:Esc];
      | I1=[Esc,Esc:0.1:30];
      | y=((k./((I.^alpha)-1))+B)*TMS;
      | Tin=[((k./((Esc.^alpha)-1))+B)*TMS,ones(1,length(I1)-1)*Tins];
      | loglog(I,y,'b');
      | hold on
      | loglog(I1,Tin,'b');
      | set(gcf, 'Position', [200 150 300 500]);
      | switch(get_param(gcb,'TCpopup1'))
      |     case 'IEC Standard Inverse'
      |         title('IEC Standard Inverse');
      |     case 'IEC Very Inverse'
      |         title('IEC Very Inverse');
      |     case 'IEC Long Time Inverse'
      |         title('IEC Long Time Inverse');
      |     case 'IEC Extremely Inverse'
      |         title('IEC Extremely Inverse');
      |      case 'IEC Ultra Inverse'
      |         title('IEC Ultra Inverse');
      |     case 'IEEE Moderately Inverse'
      |         title('IEEE Moderately Inverse');
      |     case 'IEEE Very Inverse'
      |         title('IEEE Very Inverse');
      |     case 'IEEE Extremely Inverse'
      |         title('IEEE Extremely Inverse');
      | end
      | ymax=10^ceil(log10(max(y)));
      | set(gca, 'XTick',[1:10 20]);
      | set(gca, 'YTick',[0 ymax/1000 ymax/500 ymax/200 ymax/100 ymax/50 ymax/20 ymax/10 ymax/5 ymax/2 ymax]);
      | xlim([0.9 30]);
      | ylim([0.01 ymax]);
      | xlabel(['Corriente multiplicada por Ipick-up(' num2str(PS*Vp) 'A)']);
      | ylabel('Tiempo de Operacion (Seg)');
      | grid on;
      | set(gca, 'color',[0.9608 0.9608 0.937]);
      | set(gca, 'gridcolor',[0 0.6902 0.3137]);
      mask Callback Esc1:
      | % Plotting IDMT Curve
      | clf('reset')
      | TMS = str2num(get_param(gcb,'TMS1'));
      | Vp = str2num(get_param(gcb,'Vp'));
      | PS=str2num(get_param(gcb,'PS1'));
      | k = str2num(get_param(gcb,'k1'));
      | alpha = str2num(get_param(gcb,'alpha1'));
      | B = str2num(get_param(gcb,'B1'));
      | Esc = str2num(get_param(gcb,'Esc1'));
      | Tins = str2num(get_param(gcb,'Tins1'));
      | I = [1.1:0.1:Esc];
      | I1=[Esc,Esc:0.1:30];
      | y=((k./((I.^alpha)-1))+B)*TMS;
      | Tin=[((k./((Esc.^alpha)-1))+B)*TMS,ones(1,length(I1)-1)*Tins];
      | loglog(I,y,'b');
      | hold on
      | loglog(I1,Tin,'b');
      | set(gcf, 'Position', [200 150 300 500]);
      | switch(get_param(gcb,'TCpopup1'))
      |     case 'IEC Standard Inverse'
      |         title('IEC Standard Inverse');
      |     case 'IEC Very Inverse'
      |         title('IEC Very Inverse');
      |     case 'IEC Long Time Inverse'
      |         title('IEC Long Time Inverse');
      |     case 'IEC Extremely Inverse'
      |         title('IEC Extremely Inverse');
      |      case 'IEC Ultra Inverse'
      |         title('IEC Ultra Inverse');
      |     case 'IEEE Moderately Inverse'
      |         title('IEEE Moderately Inverse');
      |     case 'IEEE Very Inverse'
      |         title('IEEE Very Inverse');
      |     case 'IEEE Extremely Inverse'
      |         title('IEEE Extremely Inverse');
      | end
      | ymax=10^ceil(log10(max(y)));
      | set(gca, 'XTick',[1:10 20]);
      | set(gca, 'YTick',[0 ymax/1000 ymax/500 ymax/200 ymax/100 ymax/50 ymax/20 ymax/10 ymax/5 ymax/2 ymax]);
      | xlim([0.9 30]);
      | ylim([0.01 ymax]);
      | xlabel(['Corriente multiplicada por Ipick-up(' num2str(PS*Vp) 'A)']);
      | ylabel('Tiempo de Operacion (Seg)');
      | grid on;
      | set(gca, 'color',[0.9608 0.9608 0.937]);
      | set(gca, 'gridcolor',[0 0.6902 0.3137]);
      mask TypeOptions TCpopup2: IEC Standard Inverse | IEC Very Inverse | IEC Long Time Inverse | IEC Extremely Inverse | IEC Ultra Inverse | IEEE Moderately Inverse | IEEE Very Inverse | IEEE Extremely Inverse
      mask Callback TCpopup2:
      | switch(get_param(gcb,'TCpopup2'))
      |     case 'IEC Standard Inverse'
      |         set_param(gcb,'k2','0.14');
      |         set_param(gcb,'alpha2','0.02');
      |         set_param(gcb,'B2','0');
      |     case 'IEC Very Inverse'
      |         set_param(gcb,'k2','13.5');
      |         set_param(gcb,'alpha2','1');
      |         set_param(gcb,'B2','0');
      |     case 'IEC Long Time Inverse'
      |         set_param(gcb,'k2','120');
      |         set_param(gcb,'alpha2','1');
      |         set_param(gcb,'B2','0');
      |     case 'IEC Extremely Inverse'
      |         set_param(gcb,'k2','80');
      |         set_param(gcb,'alpha2','2');
      |         set_param(gcb,'B2','0');
      |     case 'IEC Ultra Inverse'
      |         set_param(gcb,'k2','315.2');
      |         set_param(gcb,'alpha2','2.5');
      |         set_param(gcb,'B2','0');
      |     case 'IEEE Moderately Inverse'
      |         set_param(gcb,'k2','0.0515');
      |         set_param(gcb,'alpha2','0.02');
      |         set_param(gcb,'B2','0.114');
      |     case 'IEEE Very Inverse'
      |         set_param(gcb,'k2','19.61');
      |         set_param(gcb,'alpha2','2');
      |         set_param(gcb,'B2','0.491');
      |     case 'IEEE Extremely Inverse'
      |         set_param(gcb,'k2','28.2');
      |         set_param(gcb,'alpha2','2');
      |         set_param(gcb,'B2','0.1217');
      | end
      | % Plotting IDMT Curve
      | clf('reset')
      | TMS = str2num(get_param(gcb,'TMS2'));
      | Vp = str2num(get_param(gcb,'Vp'));
      | PS=str2num(get_param(gcb,'PS2'));
      | k = str2num(get_param(gcb,'k2'));
      | alpha = str2num(get_param(gcb,'alpha2'));
      | B = str2num(get_param(gcb,'B2'));
      | Esc = str2num(get_param(gcb,'Esc2'));
      | Tins = str2num(get_param(gcb,'Tins2'));
      | I = [1.1:0.1:Esc];
      | I1=[Esc,Esc:0.1:30];
      | y=((k./((I.^alpha)-1))+B)*TMS;
      | Tin=[((k./((Esc.^alpha)-1))+B)*TMS,ones(1,length(I1)-1)*Tins];
      | loglog(I,y,'r');
      | hold on
      | loglog(I1,Tin,'r');
      | set(gcf, 'Position', [200 150 300 500]);
      | switch(get_param(gcb,'TCpopup2'))
      |     case 'IEC Standard Inverse'
      |         title('IEC Standard Inverse');
      |     case 'IEC Very Inverse'
      |         title('IEC Very Inverse');
      |     case 'IEC Long Time Inverse'
      |         title('IEC Long Time Inverse');
      |     case 'IEC Extremely Inverse'
      |         title('IEC Extremely Inverse');
      |      case 'IEC Ultra Inverse'
      |         title('IEC Ultra Inverse');
      |     case 'IEEE Moderately Inverse'
      |         title('IEEE Moderately Inverse');
      |     case 'IEEE Very Inverse'
      |         title('IEEE Very Inverse');
      |     case 'IEEE Extremely Inverse'
      |         title('IEEE Extremely Inverse');
      | end
      | ymax=10^ceil(log10(max(y)));
      | set(gca, 'XTick',[1:10 20]);
      | set(gca, 'YTick',[0 ymax/1000 ymax/500 ymax/200 ymax/100 ymax/50 ymax/20 ymax/10 ymax/5 ymax/2 ymax]);
      | xlim([0.9 30]);
      | ylim([0.01 ymax]);
      | xlabel(['Corriente multiplicada por Ipick-up(' num2str(PS*Vp) 'A)']);
      | ylabel('Tiempo de Operacion (Seg)');
      | grid on;
      | set(gca, 'color',[0.9608 0.9608 0.937]);
      | set(gca, 'gridcolor',[0 0.6902 0.3137]);
      mask Callback PS2:
      | % Plotting IDMT Curve
      | clf('reset')
      | TMS = str2num(get_param(gcb,'TMS2'));
      | Vp = str2num(get_param(gcb,'Vp'));
      | PS=str2num(get_param(gcb,'PS2'));
      | k = str2num(get_param(gcb,'k2'));
      | alpha = str2num(get_param(gcb,'alpha2'));
      | B = str2num(get_param(gcb,'B2'));
      | Esc = str2num(get_param(gcb,'Esc2'));
      | Tins = str2num(get_param(gcb,'Tins2'));
      | I = [1.1:0.1:Esc];
      | I1=[Esc,Esc:0.1:30];
      | y=((k./((I.^alpha)-1))+B)*TMS;
      | Tin=[((k./((Esc.^alpha)-1))+B)*TMS,ones(1,length(I1)-1)*Tins];
      | loglog(I,y,'r');
      | hold on
      | loglog(I1,Tin,'r');
      | set(gcf, 'Position', [200 150 300 500]);
      | switch(get_param(gcb,'TCpopup2'))
      |     case 'IEC Standard Inverse'
      |         title('IEC Standard Inverse');
      |     case 'IEC Very Inverse'
      |         title('IEC Very Inverse');
      |     case 'IEC Long Time Inverse'
      |         title('IEC Long Time Inverse');
      |     case 'IEC Extremely Inverse'
      |         title('IEC Extremely Inverse');
      |      case 'IEC Ultra Inverse'
      |         title('IEC Ultra Inverse');
      |     case 'IEEE Moderately Inverse'
      |         title('IEEE Moderately Inverse');
      |     case 'IEEE Very Inverse'
      |         title('IEEE Very Inverse');
      |     case 'IEEE Extremely Inverse'
      |         title('IEEE Extremely Inverse');
      | end
      | ymax=10^ceil(log10(max(y)));
      | set(gca, 'XTick',[1:10 20]);
      | set(gca, 'YTick',[0 ymax/1000 ymax/500 ymax/200 ymax/100 ymax/50 ymax/20 ymax/10 ymax/5 ymax/2 ymax]);
      | xlim([0.9 30]);
      | ylim([0.01 ymax]);
      | xlabel(['Corriente multiplicada por Ipick-up(' num2str(PS*Vp) 'A)']);
      | ylabel('Tiempo de Operacion (Seg)');
      | grid on;
      | set(gca, 'color',[0.9608 0.9608 0.937]);
      | set(gca, 'gridcolor',[0 0.6902 0.3137]);
      mask Callback TMS2:
      | % Plotting IDMT Curve
      | clf('reset')
      | TMS = str2num(get_param(gcb,'TMS2'));
      | Vp = str2num(get_param(gcb,'Vp'));
      | PS=str2num(get_param(gcb,'PS2'));
      | k = str2num(get_param(gcb,'k2'));
      | alpha = str2num(get_param(gcb,'alpha2'));
      | B = str2num(get_param(gcb,'B2'));
      | Esc = str2num(get_param(gcb,'Esc2'));
      | Tins = str2num(get_param(gcb,'Tins2'));
      | I = [1.1:0.1:Esc];
      | I1=[Esc,Esc:0.1:30];
      | y=((k./((I.^alpha)-1))+B)*TMS;
      | Tin=[((k./((Esc.^alpha)-1))+B)*TMS,ones(1,length(I1)-1)*Tins];
      | loglog(I,y,'r');
      | hold on
      | loglog(I1,Tin,'r');
      | set(gcf, 'Position', [200 150 300 500]);
      | switch(get_param(gcb,'TCpopup2'))
      |     case 'IEC Standard Inverse'
      |         title('IEC Standard Inverse');
      |     case 'IEC Very Inverse'
      |         title('IEC Very Inverse');
      |     case 'IEC Long Time Inverse'
      |         title('IEC Long Time Inverse');
      |     case 'IEC Extremely Inverse'
      |         title('IEC Extremely Inverse');
      |      case 'IEC Ultra Inverse'
      |         title('IEC Ultra Inverse');
      |     case 'IEEE Moderately Inverse'
      |         title('IEEE Moderately Inverse');
      |     case 'IEEE Very Inverse'
      |         title('IEEE Very Inverse');
      |     case 'IEEE Extremely Inverse'
      |         title('IEEE Extremely Inverse');
      | end
      | ymax=10^ceil(log10(max(y)));
      | set(gca, 'XTick',[1:10 20]);
      | set(gca, 'YTick',[0 ymax/1000 ymax/500 ymax/200 ymax/100 ymax/50 ymax/20 ymax/10 ymax/5 ymax/2 ymax]);
      | xlim([0.9 30]);
      | ylim([0.01 ymax]);
      | xlabel(['Corriente multiplicada por Ipick-up(' num2str(PS*Vp) 'A)']);
      | ylabel('Tiempo de Operacion (Seg)');
      | grid on;
      | set(gca, 'color',[0.9608 0.9608 0.937]);
      | set(gca, 'gridcolor',[0 0.6902 0.3137]);
      mask Callback Tins2:
      | % Plotting IDMT Curve
      | clf('reset')
      | TMS = str2num(get_param(gcb,'TMS2'));
      | Vp = str2num(get_param(gcb,'Vp'));
      | PS=str2num(get_param(gcb,'PS2'));
      | k = str2num(get_param(gcb,'k2'));
      | alpha = str2num(get_param(gcb,'alpha2'));
      | B = str2num(get_param(gcb,'B2'));
      | Esc = str2num(get_param(gcb,'Esc2'));
      | Tins = str2num(get_param(gcb,'Tins2'));
      | I = [1.1:0.1:Esc];
      | I1=[Esc,Esc:0.1:30];
      | y=((k./((I.^alpha)-1))+B)*TMS;
      | Tin=[((k./((Esc.^alpha)-1))+B)*TMS,ones(1,length(I1)-1)*Tins];
      | loglog(I,y,'r');
      | hold on
      | loglog(I1,Tin,'r');
      | set(gcf, 'Position', [200 150 300 500]);
      | switch(get_param(gcb,'TCpopup2'))
      |     case 'IEC Standard Inverse'
      |         title('IEC Standard Inverse');
      |     case 'IEC Very Inverse'
      |         title('IEC Very Inverse');
      |     case 'IEC Long Time Inverse'
      |         title('IEC Long Time Inverse');
      |     case 'IEC Extremely Inverse'
      |         title('IEC Extremely Inverse');
      |      case 'IEC Ultra Inverse'
      |         title('IEC Ultra Inverse');
      |     case 'IEEE Moderately Inverse'
      |         title('IEEE Moderately Inverse');
      |     case 'IEEE Very Inverse'
      |         title('IEEE Very Inverse');
      |     case 'IEEE Extremely Inverse'
      |         title('IEEE Extremely Inverse');
      | end
      | ymax=10^ceil(log10(max(y)));
      | set(gca, 'XTick',[1:10 20]);
      | set(gca, 'YTick',[0 ymax/1000 ymax/500 ymax/200 ymax/100 ymax/50 ymax/20 ymax/10 ymax/5 ymax/2 ymax]);
      | xlim([0.9 30]);
      | ylim([0.01 ymax]);
      | xlabel(['Corriente multiplicada por Ipick-up(' num2str(PS*Vp) 'A)']);
      | ylabel('Tiempo de Operacion (Seg)');
      | grid on;
      | set(gca, 'color',[0.9608 0.9608 0.937]);
      | set(gca, 'gridcolor',[0 0.6902 0.3137]);
      mask Callback Esc2:
      | % Plotting IDMT Curve
      | clf('reset')
      | TMS = str2num(get_param(gcb,'TMS2'));
      | Vp = str2num(get_param(gcb,'Vp'));
      | PS=str2num(get_param(gcb,'PS2'));
      | k = str2num(get_param(gcb,'k2'));
      | alpha = str2num(get_param(gcb,'alpha2'));
      | B = str2num(get_param(gcb,'B2'));
      | Esc = str2num(get_param(gcb,'Esc2'));
      | Tins = str2num(get_param(gcb,'Tins2'));
      | I = [1.1:0.1:Esc];
      | I1=[Esc,Esc:0.1:30];
      | y=((k./((I.^alpha)-1))+B)*TMS;
      | Tin=[((k./((Esc.^alpha)-1))+B)*TMS,ones(1,length(I1)-1)*Tins];
      | loglog(I,y,'r');
      | hold on
      | loglog(I1,Tin,'r');
      | set(gcf, 'Position', [200 150 300 500]);
      | switch(get_param(gcb,'TCpopup2'))
      |     case 'IEC Standard Inverse'
      |         title('IEC Standard Inverse');
      |     case 'IEC Very Inverse'
      |         title('IEC Very Inverse');
      |     case 'IEC Long Time Inverse'
      |         title('IEC Long Time Inverse');
      |     case 'IEC Extremely Inverse'
      |         title('IEC Extremely Inverse');
      |      case 'IEC Ultra Inverse'
      |         title('IEC Ultra Inverse');
      |     case 'IEEE Moderately Inverse'
      |         title('IEEE Moderately Inverse');
      |     case 'IEEE Very Inverse'
      |         title('IEEE Very Inverse');
      |     case 'IEEE Extremely Inverse'
      |         title('IEEE Extremely Inverse');
      | end
      | ymax=10^ceil(log10(max(y)));
      | set(gca, 'XTick',[1:10 20]);
      | set(gca, 'YTick',[0 ymax/1000 ymax/500 ymax/200 ymax/100 ymax/50 ymax/20 ymax/10 ymax/5 ymax/2 ymax]);
      | xlim([0.9 30]);
      | ylim([0.01 ymax]);
      | xlabel(['Corriente multiplicada por Ipick-up(' num2str(PS*Vp) 'A)']);
      | ylabel('Tiempo de Operacion (Seg)');
      | grid on;
      | set(gca, 'color',[0.9608 0.9608 0.937]);
      | set(gca, 'gridcolor',[0 0.6902 0.3137]);
      mask TypeOptions TCpopup3: IEC Standard Inverse | IEC Very Inverse | IEC Long Time Inverse | IEC Extremely Inverse | IEC Ultra Inverse | IEEE Moderately Inverse | IEEE Very Inverse | IEEE Extremely Inverse
      mask Callback TCpopup3:
      | switch(get_param(gcb,'TCpopup3'))
      |     case 'IEC Standard Inverse'
      |         set_param(gcb,'k3','0.14');
      |         set_param(gcb,'alpha3','0.02');
      |         set_param(gcb,'B3','0');
      |     case 'IEC Very Inverse'
      |         set_param(gcb,'k3','13.5');
      |         set_param(gcb,'alpha3','1');
      |         set_param(gcb,'B3','0');
      |     case 'IEC Long Time Inverse'
      |         set_param(gcb,'k3','120');
      |         set_param(gcb,'alpha3','1');
      |         set_param(gcb,'B3','0');
      |     case 'IEC Extremely Inverse'
      |         set_param(gcb,'k3','80');
      |         set_param(gcb,'alpha3','2');
      |         set_param(gcb,'B3','0');
      |     case 'IEC Ultra Inverse'
      |         set_param(gcb,'k3','315.2');
      |         set_param(gcb,'alpha3','2.5');
      |         set_param(gcb,'B3','0');
      |     case 'IEEE Moderately Inverse'
      |         set_param(gcb,'k3','0.0515');
      |         set_param(gcb,'alpha3','0.02');
      |         set_param(gcb,'B3','0.114');
      |     case 'IEEE Very Inverse'
      |         set_param(gcb,'k3','19.61');
      |         set_param(gcb,'alpha3','2');
      |         set_param(gcb,'B3','0.491');
      |     case 'IEEE Extremely Inverse'
      |         set_param(gcb,'k3','28.2');
      |         set_param(gcb,'alpha3','2');
      |         set_param(gcb,'B3','0.1217');
      | end
      | % Plotting IDMT Curve
      | clf('reset')
      | TMS = str2num(get_param(gcb,'TMS3'));
      | Vp = str2num(get_param(gcb,'Vp'));
      | PS=str2num(get_param(gcb,'PS3'));
      | k = str2num(get_param(gcb,'k3'));
      | alpha = str2num(get_param(gcb,'alpha3'));
      | B = str2num(get_param(gcb,'B3'));
      | Esc = str2num(get_param(gcb,'Esc3'));
      | Tins = str2num(get_param(gcb,'Tins3'));
      | I = [1.1:0.1:Esc];
      | I1=[Esc,Esc:0.1:30];
      | y=((k./((I.^alpha)-1))+B)*TMS;
      | Tin=[((k./((Esc.^alpha)-1))+B)*TMS,ones(1,length(I1)-1)*Tins];
      | loglog(I,y,'m');
      | hold on
      | loglog(I1,Tin,'m');
      | set(gcf, 'Position', [200 150 300 500]);
      | switch(get_param(gcb,'TCpopup3'))
      |     case 'IEC Standard Inverse'
      |         title('IEC Standard Inverse');
      |     case 'IEC Very Inverse'
      |         title('IEC Very Inverse');
      |     case 'IEC Long Time Inverse'
      |         title('IEC Long Time Inverse');
      |     case 'IEC Extremely Inverse'
      |         title('IEC Extremely Inverse');
      |      case 'IEC Ultra Inverse'
      |         title('IEC Ultra Inverse');
      |     case 'IEEE Moderately Inverse'
      |         title('IEEE Moderately Inverse');
      |     case 'IEEE Very Inverse'
      |         title('IEEE Very Inverse');
      |     case 'IEEE Extremely Inverse'
      |         title('IEEE Extremely Inverse');
      | end
      | ymax=10^ceil(log10(max(y)));
      | set(gca, 'XTick',[1:10 20]);
      | set(gca, 'YTick',[0 ymax/1000 ymax/500 ymax/200 ymax/100 ymax/50 ymax/20 ymax/10 ymax/5 ymax/2 ymax]);
      | xlim([0.9 30]);
      | ylim([0.01 ymax]);
      | xlabel(['Corriente multiplicada por Ipick-up(' num2str(PS*Vp) 'A)']);
      | ylabel('Tiempo de Operacion (Seg)');
      | grid on;
      | set(gca, 'color',[0.9608 0.9608 0.937]);
      | set(gca, 'gridcolor',[0 0.6902 0.3137]);
      mask Callback PS3:
      | % Plotting IDMT Curve
      | clf('reset')
      | TMS = str2num(get_param(gcb,'TMS3'));
      | Vp = str2num(get_param(gcb,'Vp'));
      | PS=str2num(get_param(gcb,'PS3'));
      | k = str2num(get_param(gcb,'k3'));
      | alpha = str2num(get_param(gcb,'alpha3'));
      | B = str2num(get_param(gcb,'B3'));
      | Esc = str2num(get_param(gcb,'Esc3'));
      | Tins = str2num(get_param(gcb,'Tins3'));
      | I = [1.1:0.1:Esc];
      | I1=[Esc,Esc:0.1:30];
      | y=((k./((I.^alpha)-1))+B)*TMS;
      | Tin=[((k./((Esc.^alpha)-1))+B)*TMS,ones(1,length(I1)-1)*Tins];
      | loglog(I,y,'m');
      | hold on
      | loglog(I1,Tin,'m');
      | set(gcf, 'Position', [200 150 300 500]);
      | switch(get_param(gcb,'TCpopup3'))
      |     case 'IEC Standard Inverse'
      |         title('IEC Standard Inverse');
      |     case 'IEC Very Inverse'
      |         title('IEC Very Inverse');
      |     case 'IEC Long Time Inverse'
      |         title('IEC Long Time Inverse');
      |     case 'IEC Extremely Inverse'
      |         title('IEC Extremely Inverse');
      |      case 'IEC Ultra Inverse'
      |         title('IEC Ultra Inverse');
      |     case 'IEEE Moderately Inverse'
      |         title('IEEE Moderately Inverse');
      |     case 'IEEE Very Inverse'
      |         title('IEEE Very Inverse');
      |     case 'IEEE Extremely Inverse'
      |         title('IEEE Extremely Inverse');
      | end
      | ymax=10^ceil(log10(max(y)));
      | set(gca, 'XTick',[1:10 20]);
      | set(gca, 'YTick',[0 ymax/1000 ymax/500 ymax/200 ymax/100 ymax/50 ymax/20 ymax/10 ymax/5 ymax/2 ymax]);
      | xlim([0.9 30]);
      | ylim([0.01 ymax]);
      | xlabel(['Corriente multiplicada por Ipick-up(' num2str(PS*Vp) 'A)']);
      | ylabel('Tiempo de Operacion (Seg)');
      | grid on;
      | set(gca, 'color',[0.9608 0.9608 0.937]);
      | set(gca, 'gridcolor',[0 0.6902 0.3137]);
      mask Callback TMS3:
      | % Plotting IDMT Curve
      | clf('reset')
      | TMS = str2num(get_param(gcb,'TMS3'));
      | Vp = str2num(get_param(gcb,'Vp'));
      | PS=str2num(get_param(gcb,'PS3'));
      | k = str2num(get_param(gcb,'k3'));
      | alpha = str2num(get_param(gcb,'alpha3'));
      | B = str2num(get_param(gcb,'B3'));
      | Esc = str2num(get_param(gcb,'Esc3'));
      | Tins = str2num(get_param(gcb,'Tins3'));
      | I = [1.1:0.1:Esc];
      | I1=[Esc,Esc:0.1:30];
      | y=((k./((I.^alpha)-1))+B)*TMS;
      | Tin=[((k./((Esc.^alpha)-1))+B)*TMS,ones(1,length(I1)-1)*Tins];
      | loglog(I,y,'m');
      | hold on
      | loglog(I1,Tin,'m');
      | set(gcf, 'Position', [200 150 300 500]);
      | switch(get_param(gcb,'TCpopup3'))
      |     case 'IEC Standard Inverse'
      |         title('IEC Standard Inverse');
      |     case 'IEC Very Inverse'
      |         title('IEC Very Inverse');
      |     case 'IEC Long Time Inverse'
      |         title('IEC Long Time Inverse');
      |     case 'IEC Extremely Inverse'
      |         title('IEC Extremely Inverse');
      |      case 'IEC Ultra Inverse'
      |         title('IEC Ultra Inverse');
      |     case 'IEEE Moderately Inverse'
      |         title('IEEE Moderately Inverse');
      |     case 'IEEE Very Inverse'
      |         title('IEEE Very Inverse');
      |     case 'IEEE Extremely Inverse'
      |         title('IEEE Extremely Inverse');
      | end
      | ymax=10^ceil(log10(max(y)));
      | set(gca, 'XTick',[1:10 20]);
      | set(gca, 'YTick',[0 ymax/1000 ymax/500 ymax/200 ymax/100 ymax/50 ymax/20 ymax/10 ymax/5 ymax/2 ymax]);
      | xlim([0.9 30]);
      | ylim([0.01 ymax]);
      | xlabel(['Corriente multiplicada por Ipick-up(' num2str(PS*Vp) 'A)']);
      | ylabel('Tiempo de Operacion (Seg)');
      | grid on;
      | set(gca, 'color',[0.9608 0.9608 0.937]);
      | set(gca, 'gridcolor',[0 0.6902 0.3137]);
      mask Callback Tins3:
      | % Plotting IDMT Curve
      | clf('reset')
      | TMS = str2num(get_param(gcb,'TMS3'));
      | Vp = str2num(get_param(gcb,'Vp'));
      | PS=str2num(get_param(gcb,'PS3'));
      | k = str2num(get_param(gcb,'k3'));
      | alpha = str2num(get_param(gcb,'alpha3'));
      | B = str2num(get_param(gcb,'B3'));
      | Esc = str2num(get_param(gcb,'Esc3'));
      | Tins = str2num(get_param(gcb,'Tins3'));
      | I = [1.1:0.1:Esc];
      | I1=[Esc,Esc:0.1:30];
      | y=((k./((I.^alpha)-1))+B)*TMS;
      | Tin=[((k./((Esc.^alpha)-1))+B)*TMS,ones(1,length(I1)-1)*Tins];
      | loglog(I,y,'m');
      | hold on
      | loglog(I1,Tin,'m');
      | set(gcf, 'Position', [200 150 300 500]);
      | switch(get_param(gcb,'TCpopup3'))
      |     case 'IEC Standard Inverse'
      |         title('IEC Standard Inverse');
      |     case 'IEC Very Inverse'
      |         title('IEC Very Inverse');
      |     case 'IEC Long Time Inverse'
      |         title('IEC Long Time Inverse');
      |     case 'IEC Extremely Inverse'
      |         title('IEC Extremely Inverse');
      |      case 'IEC Ultra Inverse'
      |         title('IEC Ultra Inverse');
      |     case 'IEEE Moderately Inverse'
      |         title('IEEE Moderately Inverse');
      |     case 'IEEE Very Inverse'
      |         title('IEEE Very Inverse');
      |     case 'IEEE Extremely Inverse'
      |         title('IEEE Extremely Inverse');
      | end
      | ymax=10^ceil(log10(max(y)));
      | set(gca, 'XTick',[1:10 20]);
      | set(gca, 'YTick',[0 ymax/1000 ymax/500 ymax/200 ymax/100 ymax/50 ymax/20 ymax/10 ymax/5 ymax/2 ymax]);
      | xlim([0.9 30]);
      | ylim([0.01 ymax]);
      | xlabel(['Corriente multiplicada por Ipick-up(' num2str(PS*Vp) 'A)']);
      | ylabel('Tiempo de Operacion (Seg)');
      | grid on;
      | set(gca, 'color',[0.9608 0.9608 0.937]);
      | set(gca, 'gridcolor',[0 0.6902 0.3137]);
      mask Callback Esc3:
      | % Plotting IDMT Curve
      | clf('reset')
      | TMS = str2num(get_param(gcb,'TMS3'));
      | Vp = str2num(get_param(gcb,'Vp'));
      | PS=str2num(get_param(gcb,'PS3'));
      | k = str2num(get_param(gcb,'k3'));
      | alpha = str2num(get_param(gcb,'alpha3'));
      | B = str2num(get_param(gcb,'B3'));
      | Esc = str2num(get_param(gcb,'Esc3'));
      | Tins = str2num(get_param(gcb,'Tins3'));
      | I = [1.1:0.1:Esc];
      | I1=[Esc,Esc:0.1:30];
      | y=((k./((I.^alpha)-1))+B)*TMS;
      | Tin=[((k./((Esc.^alpha)-1))+B)*TMS,ones(1,length(I1)-1)*Tins];
      | loglog(I,y,'m');
      | hold on
      | loglog(I1,Tin,'m');
      | set(gcf, 'Position', [200 150 300 500]);
      | switch(get_param(gcb,'TCpopup3'))
      |     case 'IEC Standard Inverse'
      |         title('IEC Standard Inverse');
      |     case 'IEC Very Inverse'
      |         title('IEC Very Inverse');
      |     case 'IEC Long Time Inverse'
      |         title('IEC Long Time Inverse');
      |     case 'IEC Extremely Inverse'
      |         title('IEC Extremely Inverse');
      |      case 'IEC Ultra Inverse'
      |         title('IEC Ultra Inverse');
      |     case 'IEEE Moderately Inverse'
      |         title('IEEE Moderately Inverse');
      |     case 'IEEE Very Inverse'
      |         title('IEEE Very Inverse');
      |     case 'IEEE Extremely Inverse'
      |         title('IEEE Extremely Inverse');
      | end
      | ymax=10^ceil(log10(max(y)));
      | set(gca, 'XTick',[1:10 20]);
      | set(gca, 'YTick',[0 ymax/1000 ymax/500 ymax/200 ymax/100 ymax/50 ymax/20 ymax/10 ymax/5 ymax/2 ymax]);
      | xlim([0.9 30]);
      | ylim([0.01 ymax]);
      | xlabel(['Corriente multiplicada por Ipick-up(' num2str(PS*Vp) 'A)']);
      | ylabel('Tiempo de Operacion (Seg)');
      | grid on;
      | set(gca, 'color',[0.9608 0.9608 0.937]);
      | set(gca, 'gridcolor',[0 0.6902 0.3137]);
      mask DialogControl Container6 Prompt: Protecciones
      mask DialogControl Container8 Prompt: Topologia 1
      mask DialogControl Container9 Prompt: Proteccion 51
      mask DialogControl Container10 Prompt: Proteccion 50
      mask DialogControl Container8_copy Prompt: Topologia 2
      mask DialogControl Container9_copy Prompt: Proteccion 51
      mask DialogControl Container10_copy Prompt: Proteccion 50
      mask DialogControl Container8_copy_copy Prompt: Topologia 3
      mask DialogControl Container9_copy_copy Prompt: Proteccion 51
      mask DialogControl Container10_copy_copy Prompt: Proteccion 50
      mask DialogControl Container17 Prompt: Caracteristicas Trafo Corriente
      mask Display:
      | port_label('input',1,'D');
      | port_label('input',2,'I');
      | port_label('output',1,'S');
      | text(0.62, 0.5,'50', 'horizontalAlignment', 'center');
      | text(0.62, 0.3,'51', 'horizontalAlignment', 'center');
      | plot([0.08:0.01:0.32]+0.4,[0:0.01:0.24]*0+0.40);
      | plot(0.25*sin([0:pi/20:2*pi])+0.6,0.25*cos([0:pi/20:2*pi])+0.4);
      | %Linea Salida
      | plot([0.85:0.01:1],[0:0.01:0.15]*0+0.4);
      | %Linea Corriente
      | plot([0.2:0.01:0.35],[0:0.01:0.15]*0+0.4);
      | plot([0.1:0.01:0.2],[0:0.01:0.1]*0+0.15);
      | plot([0.1:0.01:0.35]*0+0.2,[0:0.01:0.25]+0.15);
      | %Linea tension
      | plot([0.15:0.01:0.6],[0:0.01:0.45]*0+0.7);
      | plot([0:0.01:0.05]*0+0.6,[0:0.01:0.05]+0.65);
  RE : powerlib/Electrical Sources/Three-Phase Source  InternalConnection=Yg  VoltagePhases=off  Voltage=13200  PhaseAngle=0  Voltage_phases=[25e3 25e3 25e3]/sqrt(3)  PhaseAngles_phases=[0 -120 +120]  Frequency=60  NonIdealSource=on  SpecifyImpedance=on  Resistance=25^2/1000/10  Inductance=25^2/1000/377  ShortCircuitLevel=277e6  BaseVoltage=13200  XRratio=10  BusType=swing  Pref=10e3  Qref=0  Prefabc=[10e3, 10e3, 10e3]  Qrefabc=[0, 0, 0]  Qmin=-inf  Qmax=inf
  SW1 : powerlib/Elements/Three-Phase Breaker  InitialState=closed  SwitchA=on  SwitchB=on  SwitchC=on  SwitchTimes=1000000000  External=on  BreakerResistance=0.001  SnubberResistance=1e6  SnubberCapacitance=inf  Measurements=None
      link override Breaker A: Measurements=None
      link override Breaker B: Measurements=None
      link override Breaker C: Measurements=None
  SW2 : powerlib/Elements/Three-Phase Breaker  InitialState=closed  SwitchA=on  SwitchB=on  SwitchC=on  SwitchTimes=1000000000  External=on  BreakerResistance=0.001  SnubberResistance=1e6  SnubberCapacitance=inf  Measurements=None
      link override Breaker A: Measurements=None
      link override Breaker B: Measurements=None
      link override Breaker C: Measurements=None
  Scope5 : Scope  NumInputPorts=3
  Scope8 : Scope
  Scope9 : Scope
  Step1 : Step  Time=0.1  Before=1  After=0  SampleTime=0
  Step2 : Step  Time=10  Before=1  After=0  SampleTime=0
  Subsystem : Subsystem
  Switch4 : Switch  Criteria=u2 ~= 0
  To Workspace : ToWorkspace  VariableName=datos_grafica  SaveFormat=Structure With Time  SampleTime=-1
  UCL : Subsystem  mask(Selector de configuración de red eléctrica){modo=Automática, manual=Distribuida}
      mask help: Bloque diseñado para variar la configuración de la unidad central de control para la configuración manual y automática.
      mask TypeOptions modo: Automática | Manual
      mask Callback modo:
      | h1 = getSimulinkBlockHandle(gcb);
      | modo = get_param(h1,'modo');
      | if strcmp(modo,'Automática')
      |     Vuc=1;
      |     set_param(h1,'MaskVisibilities',{'on','off'});
      |     man=0;
      | elseif strcmp(modo,'Manual')
      |     Vuc=0;
      |     set_param(h1,'MaskVisibilities',{'on','on'});
      | end
      mask TypeOptions manual: Radial | Isla | Distribuida
      mask Callback manual:
      | clc,
      | h2 = getSimulinkBlockHandle(gcb);
      | manuales = get_param(h2,'manual');
      | if strcmp(manuales,'Radial')
      |     man=1;
      | elseif strcmp(manuales,'Isla')
      |     man=2;
      | elseif strcmp(manuales,'Distribuida')
      |     man=3;
      | end
      mask DialogControl ParameterGroupVar Prompt: Selección del tipo de configuración de la red eléctrica
      mask Display:
      | color('black');disp('UCL');
      | color('blue');
      | port_label('input',1,'Medida_RE');
      | port_label('input',2,'Medida_GD');
      | color('red');
      | port_label('output',1,'Config');
  powergui : powerlib/powergui  Priority=1  SimulationMode=Discrete  SampleTime=Ts  frequency=60  Iterations=50  frequencyindice=0  Pbase=100e6  ErrMax=1e-4  UnitsV=kV  UnitsW=MW  buscounter=0  FunctionMessages=off  echomessages=off  EnableUseOfTLC=off  CurrentSourceSwitches=on  DisableSnubberDevices=off  DisableRonSwitches=off  DisableVfSwitches=off  DisplayEquations=off  SolverType=Tustin/Backward Euler (TBE)  Interpol=off  ExternalGateDelay=off  methode=off  Ts=10  x0status=blocks  SPID=off  SwTol=0  HookPort=off  RestoreLinks=warning  ResistiveCurrentMeasurement=off  Frange=[0:2:500]  Ylog=off  Xlog=on  ShowGrid=off  save=off  variable=ZData  structure=0  ZoomFFT=off  StartTime=0.0  cycles=1  DisplayStyle=1  fundamental=60  FreqAxis=off  MaxFrequency=1000  frequencyindicesteady=1  RmsSteady=1  display=off
  wires:
  M-P2/1 -> [M_P2]
  Step1/1 -> SW1/1
  Step2/1 -> SW2/1
  [I_P3] -> Scope5/3
  [I_P2] -> Scope5/2
  [I_P1] -> Scope5/1
  [M_P1] -> Mux1/1
  Mux1/1 -> To Workspace/1, Scope8/1
  [M_P2] -> Mux1/2
  [M_P1] -> UCL/1(RED)
  [M_P2] -> UCL/2(GD)
  [Config] -> Mux1/3
  [Config] -> RB1/1(En)
  [Config] -> R3/1(En)
  [I_P1] -> RB1/2(I)
  [I_P3] -> R3/2(I)
  R3/1(Trip) -> INTERRUPTOR R3/1
  RB1/1(Trip) -> INTERRUPTOR R1/1
  EMISOR-RECEPTOR/1 -> Display9/1, Subsystem/Trigger
  EMISOR-RECEPTOR/2 -> Mux3/2, Bus B2 M4/1, Display10/1
  [CON_R_R2] -> Logical Operator/1
  UCL/1(CONTROL) -> Display14/1, Switch4/2, Switch4/1
  Switch4/1 -> Display13/1, [Config], Scope9/1
  Configuración inicial4/1 -> Switch4/3
  Logical Operator/1 -> INTERRUPTOR R2/1
  Subsystem/1(Out1) -> Bus B2 M3/1, [CON_R_R2], Mux3/1
  Mux2/1 -> Bus B2 M1/1
  [M_P2] -> EMISOR-RECEPTOR/1, Bus B2 M6/1
  Mux3/1 -> Bus B2 M2/1
  Configuración inicial1/1 -> Goto1/1
  [I_P2] -> Mux2/2
  P1/1 -> [I_P1], M-P1/1
  M-P1/1 -> [M_P1]
  P2/1 -> [I_P2], M-P2/1
  P3/1 -> [I_P3]
  [M_P2] -> Mux2/1
  connections:
  RE/RConn3 -- SW1/LConn3
  RE/RConn2 -- SW1/LConn2
  RE/RConn1 -- SW1/LConn1
  P1/LConn1 -- SW1/RConn1
  P2/LConn3 -- SW2/RConn3
  P2/LConn2 -- SW2/RConn2
  P2/LConn1 -- SW2/RConn1
  GD/RConn1 -- SW2/LConn1
  GD/RConn2 -- SW2/LConn2
  GD/RConn3 -- SW2/LConn3
  INTERRUPTOR R3/RConn1 -- P4/LConn1
  INTERRUPTOR R3/RConn2 -- P4/LConn2
  INTERRUPTOR R3/RConn3 -- P4/LConn3
  "               LF-1"/LConn3 -- Carga 1/LConn3 -- INTERRUPTOR R2/RConn3 -- P3/RConn3 -- INTERRUPTOR R3/LConn3
  SW1/RConn3 -- P1/LConn3
  P1/RConn1 -- INTERRUPTOR R1/LConn1
  P1/RConn2 -- INTERRUPTOR R1/LConn2
  P1/RConn3 -- INTERRUPTOR R1/LConn3
  P2/RConn3 -- INTERRUPTOR R2/LConn3
  P2/RConn2 -- INTERRUPTOR R2/LConn2
  P2/RConn1 -- INTERRUPTOR R2/LConn1
  P4/RConn1 -- Carga 2/LConn1
  P4/RConn2 -- Carga 2/LConn2
  P4/RConn3 -- Carga 2/LConn3
  "               LF-1"/LConn1 -- INTERRUPTOR R2/RConn1 -- INTERRUPTOR R3/LConn1 -- P3/RConn1 -- Carga 1/LConn1
  "               LF-1"/LConn2 -- INTERRUPTOR R2/RConn2 -- P3/RConn2 -- INTERRUPTOR R3/LConn2 -- Carga 1/LConn2
  P1/LConn2 -- SW1/RConn2
  P3/LConn2 -- INTERRUPTOR R1/RConn2
  INTERRUPTOR R1/RConn3 -- P3/LConn3
  INTERRUPTOR R1/RConn1 -- P3/LConn1
